simulink model "IEEE34bus_v2019b_Phasor_DPL"  (R2019b)
settings: Solver=VariableStepAuto  StartTime=0.0  StopTime=100  FixedStep=Ts  RelTol=1e-3
InitFcn:
  | a=1; % Loading Factor
  | Ts=0.1;% For Delay Blocks in Voltage Regulator Controls
  | 
  | % Simulation data for the IEEE 34 Node Test Feeder model
  | mi2km = 1.60934;%  miles to km conversion
  | ft2km = 0.0003048; % feet to km conversion
  | ms2F = 1*1e-6/(2*pi*60);% microsiemens to Farads conversion
  | 
  | %% Configuration 300 - series reactance - ohm/mile
  | R_300 = [1.3368 0.2101 0.2130;0.2101 1.3238 0.2066;0.2130 0.2066 1.3294];
  | X_300 = [1.3343 0.5779 0.5015;0.5779 1.3569 0.4591;0.5015 0.4591 1.3471];
  | % charging susceptance - microsiemens/mile
  | B_300 = [5.3350 -1.5313 -0.9943;-1.5313 5.0979 -0.6212;-0.9943 -0.6212 4.8880];
  | 
  | R_300 = R_300/mi2km;
  | L_300 = (X_300/(2*pi*60))/mi2km;
  | C_300 =(B_300*ms2F)/mi2km;
  | 
  | %% Configuration 301 - series reactance - ohm/mile
  | R_301 = [1.9300 0.2327 0.2359;0.2327 1.9157 0.2288;0.2359 0.2288 1.9219];
  | X_301 = [1.4115 0.6442 0.5691;0.6442 1.4281 0.5238;0.5691 0.5238 1.4209];
  | % charging susceptance - microsiemens/mile
  | B_301 = [5.1207 -1.4364 -0.9402;-1.4364 4.9055 -0.5951;-0.9402 -0.5951 4.7154];
  | 
  | R_301 = R_301/mi2km;
  | L_301 = (X_301/(2*pi*60))/mi2km;
  | C_301 =(B_301*ms2F)/mi2km;
  | 
  | 
  | %% Configuration 302 - series reactance - ohm/mile
  | R_302 = [2.7995 0 0;0 0 0;0 0 0];
  | X_302 = [1.4855 0 0;0 0 0;0 0 0];
  | % charging susceptance - microsiemens/mile
  | B_302 = [4.2251 0 0;0 0 0;0 0 0];
  | 
  | R_302 = R_302/mi2km;
  | L_302 = (X_302/(2*pi*60))/mi2km;
  | C_302 =(B_302*ms2F)/mi2km;
  | 
  | %% Configuration 303 - series reactance - ohm/mile
  | R_303 = [0 0 0;0 2.7995 0;0 0 0];
  | X_303 = [0 0 0;0 1.4855 0;0 0 0];
  | % charging susceptance - microsiemens/mile
  | B_303 = [0 0 0;0 4.2251 0;0 0 0];
  | 
  | R_303 = R_303/mi2km;
  | L_303 = (X_303/(2*pi*60))/mi2km;
  | C_303 =(B_303*ms2F)/mi2km;
  | 
  | %% Configuration 303 - series reactance - ohm/mile
  | R_304 = [0 0 0;0 1.9217 0;0 0 0];
  | X_304 = [0 0 0;0 1.4212 0;0 0 0];
  | % charging susceptance - microsiemens/mile
  | B_304 = [0 0 0;0 4.3637 0;0 0 0];
  | 
  | R_304 = R_304/mi2km;
  | L_304 = (X_304/(2*pi*60))/mi2km;
  | C_304 =(B_304*ms2F)/mi2km;
undefined symbols (not defined in the file or in its folder): find_system, j
libraries: powerlib x239, powerlib_meascontrol x22
(part 1 of 4)
settings Model: ARTEMISmethode_block_infos=$$__separator__$$pi34variableloadwith3PV/ARTEMIS Guide$$__separator__$$  Creator=Arun  LastModifiedBy=USARSUR
settings SolverCC: ShapePreserveControl=EnableAll  SolverResetMethod=Robust
settings DataIOCC: ReturnWorkspaceOutputs=off
settings DebuggingCC: UnconnectedInputMsg=none  UnconnectedOutputMsg=none  UnconnectedLineMsg=none  ArithmeticOperatorsInVariantConditions=warning
settings SFSimCC: SimUseLocalCustomCode=off  CustomCodeUndefinedFunction=UseInterfaceOnly
settings RTWCC: RTWUseLocalCustomCode=off
settings CodeAppCC: StateflowObjectComments=on
settings SimscapeCC: SimscapeNormalizeSystem=off

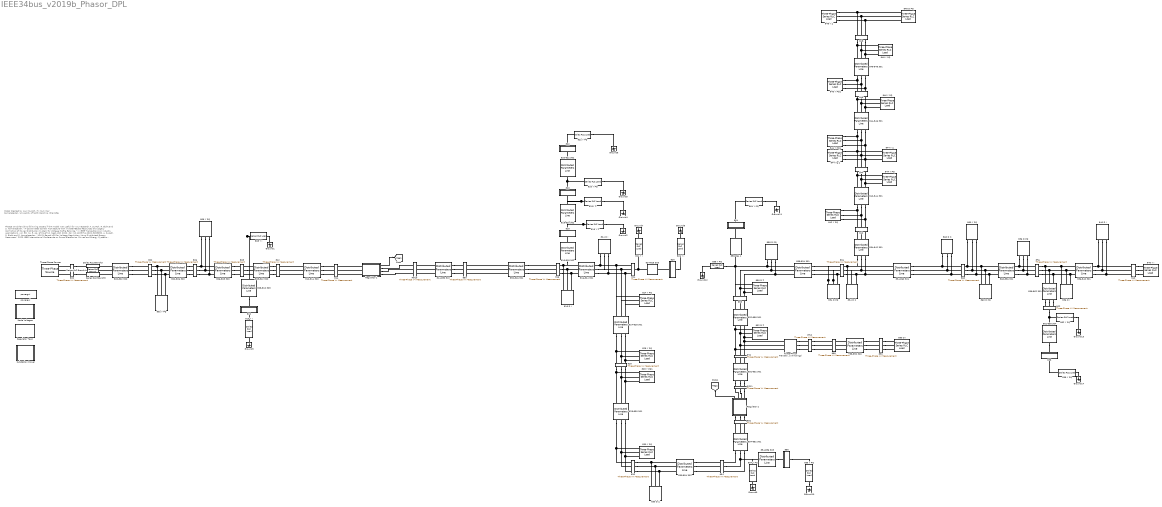
== system IEEE34bus_v2019b_Phasor_DPL ==
  note: Model Created by
      | Arun Suresh, Dr. Sukumar Kamalasadan,
      | University of North Carolina, Charlotte
  note: Please consider citing following papers if the model was useful for your research
      |
      | A. Suresh, R. Bisht and S. Kamalasadan, "A Coordinated Control Architecture With Inverter-Based Resources and Legacy
      | Controllers of Power Distribution System for Voltage Profile Balance," in IEEE Transactions on Industry Applications, vol. 58,
      | no. 5, pp. 6701-6712, Sept.-Oct. 2022, doi: 10.1109/TIA.2022.3183030.
      |
      | A. Suresh, R. Bisht and S. Kamalasadan, "ADMM Based LQR for Voltage Regulation Using Distributed Energy Resources,"
      | 2020 IEEE International Conference on Power Electronics, Drives and Energy Systems (PEDES), 2020, pp. 1-6,
      | doi: 10.1109/PEDES49360.2020.9379625.
  800 : powerlib/Measurements/Three-Phase V-I Measurement  VoltageMeasurement=phase-to-ground  SetLabelV=on  LabelV=V800  Vpu=off  VpuLL=off  CurrentMeasurement=yes  SetLabelI=on  LabelI=I800  Ipu=off  Pbase=100e6  Vbase=24900  OutputType=Complex  PhasorSimulation=on  PSBequivalent=0
      settings: SourceProductName=Simscape Electrical
  800-802 300 : powerlib/Elements/Distributed Parameters Line  Phases=3  Frequency=60  Resistance=R_300  Inductance=L_300  Capacitance=C_300  Length=2580*ft2km  x1=[1249.92473603846 26131.3609955303 26008.9539859825;376.991118430775 376.991118430775 376.991118430775;1.94160409252664 0.298080510916726 1.87234887562591]  x2=[1259.05409163765 26090.5936404474 25972.8081204705;376.991118430775 376.991118430775 376.991118430775;1.94853386735394 0.297367964044877 1.87140996339877]  x3=[10.8891002568441 16.0809137174944 5.85414031081314;376.991118430775 376.991118430775 376.991118430775;1.79537229650244 1.0798554030988 3.0143696476072]  x4=[7.9005802428278 145.280765286366 127.082333761023;376.991118430775 376.991118430775 376.991118430775;-1.40330022719033 0.219032441235353 1.82940682644033]  x5=3.46223763231864e-06  V1=[1250 2.613e+04 2.601e+04;377 377 377;1.942 0.2981 1.872]  V2=[1266 2.604e+04 2.593e+04;377 377 377;1.957 0.2977 1.871]  I1=[20.27 83.58 67.93;377 377 377;1.911 2.489 -2.004]  I2=[17.23 215.7 185.4;377 377 377;-1.237 -0.02332 1.623]  nHarmo=1  Measurements=None
      settings: SourceProductName=Simscape Power Systems
  802 : powerlib/Measurements/Three-Phase V-I Measurement  VoltageMeasurement=phase-to-ground  SetLabelV=on  LabelV=V802  Vpu=off  VpuLL=off  CurrentMeasurement=yes  SetLabelI=on  LabelI=I802  Ipu=off  Pbase=100e6  Vbase=24900  OutputType=Complex  PhasorSimulation=on  PSBequivalent=0
      settings: SourceProductName=Simscape Electrical
  802 Y PQ : powerlib/Elements/Three-Phase Series RLC Load  LConnTagsString=A|B|C  Configuration=Y (grounded)  NominalVoltage=1000  Vabc=[ 1.0 1.0 1.0]*14376.02  Vabcp=[1e3 1e3 1e3]  NominalFrequency=60  UnbalancedPower=on  ActivePower=10e3  InductivePower=100  CapacitivePower=100  Pabc="[1e-3  30 25]*1e3/2 *a"  QLabc=[0 15 14]*1e3/2 *a  QCabc=[0 0 0]  Pabcp=[10e3 9e3 11e3]  QLabcp=[100 90 110]  QCabcp=[100 90 110]  Measurements=None  LoadType=constant PQ
      settings: SourceProductName=Simscape Electrical
  802-806 300 : powerlib/Elements/Distributed Parameters Line  Phases=3  Frequency=60  Resistance=R_300  Inductance=L_300  Capacitance=C_300  Length=1730*ft2km  x1=[1259.05409163765 26090.5936404474 25972.8081204705;376.991118430775 376.991118430775 376.991118430775;1.94896388592436 0.297734464671701 1.87176932780632]  x2=[1265.00206352771 26063.5744788682 25949.4488445243;376.991118430775 376.991118430775 376.991118430775;1.9541920214162 0.297265793458538 1.87113645272041]  x3=[11.3930334018987 16.7161727751993 5.49036931474212;376.991118430775 376.991118430775 376.991118430775;1.8672823424592 1.04909387427718 2.69761493179715]  x4=[8.35366973653815 144.343309301947 125.639738686776;376.991118430775 376.991118430775 376.991118430775;-1.30493901718946 0.217938427430677 1.83893721530045]  x5=2.32157794725242e-06  V1=[1266 2.604e+04 2.593e+04;377 377 377;1.958 0.2981 1.872]  V2=[1276 2.597e+04 2.587e+04;377 377 377;1.969 0.2978 1.871]  I1=[20.86 83.31 66.2;377 377 377;1.948 2.482 -2.001]  I2=[17.78 214.8 183.7;377 377 377;-1.196 -0.02508 1.628]  nHarmo=1  Measurements=None
      settings: SourceProductName=Simscape Power Systems
  806 : powerlib/Measurements/Three-Phase V-I Measurement  VoltageMeasurement=phase-to-ground  SetLabelV=on  LabelV=V806  Vpu=off  VpuLL=off  CurrentMeasurement=yes  SetLabelI=on  LabelI=I806  Ipu=off  Pbase=100e6  Vbase=24900  OutputType=Complex  PhasorSimulation=on  PSBequivalent=0
      settings: SourceProductName=Simscape Electrical
  806 Y PQ : powerlib/Elements/Three-Phase Series RLC Load  LConnTagsString=A|B|C  Configuration=Y (grounded)  NominalVoltage=1000  Vabc=[ 1.0 1.0 1.0]*14376.02  Vabcp=[1e3 1e3 1e3]  NominalFrequency=60  UnbalancedPower=on  ActivePower=10e3  InductivePower=100  CapacitivePower=100  Pabc="[1e-3  30 25]*1e3/2 *a"  QLabc=[0 15 14]*1e3/2 *a  QCabc=[0 0 0]  Pabcp=[10e3 9e3 11e3]  QLabcp=[100 90 110]  QCabcp=[100 90 110]  Measurements=None  LoadType=constant PQ
      settings: SourceProductName=Simscape Electrical
  806-808 300 : powerlib/Elements/Distributed Parameters Line  Phases=3  Frequency=60  Resistance=R_300  Inductance=L_300  Capacitance=C_300  Length=32230*ft2km  x1=[1265.00206352771 26063.5744788682 25949.4488445243;376.991118430775 376.991118430775 376.991118430775;1.93876194330106 0.284114888613696 1.85824161221398]  x2=[1379.02773374669 25564.6834715686 25530.0919618854;376.991118430775 376.991118430775 376.991118430775;2.03883042540818 0.275533008845952 1.84631857982753]  x3=[11.8723696066793 16.932587213612 5.46705259706118;376.991118430775 376.991118430775 376.991118430775;1.91664860231484 1.0200357742312 2.37957123806189]  x4=[8.71372797948738 140.351675369273 121.993071750806;376.991118430775 376.991118430775 376.991118430775;-1.24897193669699 0.190805225356627 1.82267186347869]  x5=4.32511313525697e-05  V1=[1276 2.597e+04 2.587e+04;377 377 377;1.953 0.2847 1.858]  V2=[1495 2.48e+04 2.487e+04;377 377 377;2.136 0.2802 1.845]  I1=[21.34 82.37 64.1;377 377 377;1.967 2.465 -2.009]  I2=[18.04 208.6 178.4;377 377 377;-1.188 -0.05185 1.608]  nHarmo=1  Measurements=None
      settings: SourceProductName=Simscape Power Systems
  808 : powerlib/Measurements/Three-Phase V-I Measurement  VoltageMeasurement=phase-to-ground  SetLabelV=on  LabelV=V808  Vpu=off  VpuLL=off  CurrentMeasurement=yes  SetLabelI=on  LabelI=I808  Ipu=off  Pbase=100e6  Vbase=24900  OutputType=Complex  PhasorSimulation=on  PSBequivalent=0
      settings: SourceProductName=Simscape Electrical
  808 Y I : powerlib/Elements/Series RLC Load  LConnTagsString=a  RConnTagsString=__new0  NominalVoltage=1.0*14376.02  NominalFrequency=60  ActivePower=16e3/2*a  InductivePower=8e3/2*a  CapacitivePower=0  Setx0=off  InitialVoltage=0  SetiL0=off  InitialCurrent=0  Measurements=None  LoadType=constant I
      settings: SourceProductName=Simscape Electrical
  808-810 303 : powerlib/Elements/Distributed Parameters Line  Phases=1  Frequency=60  Resistance=R_303(2,2)  Inductance=L_303(2,2)  Capacitance=C_303(2,2)  Length=5804*ft2km  x1=[20983.741763622;376.991118430775;-2.11327141774278]  x2=[20980.659007782;376.991118430775;-2.11328221150665]  x3=[34.4426323640272;376.991118430775;-2.10433384251084]  x4=[36.0584227611352;376.991118430775;-2.12451473195879]  x5=7.30496713110932e-06  V1=[2.049e+04;377;-2.115]  V2=[2.048e+04;377;-2.115]  I1=[33.62;377;-2.106]  I2=[35.2;377;-2.126]  nHarmo=1  Measurements=None
      settings: SourceProductName=Simscape Power Systems
  808-812 300 : powerlib/Elements/Distributed Parameters Line  Phases=3  Frequency=60  Resistance=R_300  Inductance=L_300  Capacitance=C_300  Length=37500*ft2km  x1=[1379.02773374669 25564.6834715686 25530.0919618854;376.991118430775 376.991118430775 376.991118430775;2.03616431027156 0.273260704959647 1.84409052050068]  x2=[1508.53935989797 24986.4688915968 25049.8377706755;376.991118430775 376.991118430775 376.991118430775;2.14075084651696 0.263537048880938 1.82978913917078]  x3=[11.7784392805967 17.0338463877836 4.39298540674719;376.991118430775 376.991118430775 376.991118430775;2.01811649155585 1.07121274431336 2.29220318868309]  x4=[8.3337594581597 137.573158671839 120.282432485824;376.991118430775 376.991118430775 376.991118430775;-1.14964617525409 0.170446005290606 1.81272355740158]  x5=5.03232213999802e-05  V1=[1495 2.48e+04 2.487e+04;377 377 377;2.133 0.2779 1.843]  V2=[1780 2.344e+04 2.372e+04;377 377 377;2.292 0.2729 1.827]  I1=[21.39 84.55 65.08;377 377 377;2.029 2.481 -1.979]  I2=[17.55 204.1 175.2;377 377 377;-1.153 -0.07064 1.596]  nHarmo=1  Measurements=None
      settings: SourceProductName=Simscape Power Systems
  810 : Subsystem
  810 Y I : powerlib/Elements/Series RLC Load  LConnTagsString=a  RConnTagsString=__new0  NominalVoltage=1.0*14376.02  NominalFrequency=60  ActivePower=16e3/2*a  InductivePower=8e3/2*a  CapacitivePower=0  Setx0=off  InitialVoltage=0  SetiL0=off  InitialCurrent=0  Measurements=None  LoadType=constant I
      settings: SourceProductName=Simscape Electrical
  812 : powerlib/Measurements/Three-Phase V-I Measurement  VoltageMeasurement=phase-to-ground  SetLabelV=on  LabelV=V812  Vpu=off  VpuLL=off  CurrentMeasurement=yes  SetLabelI=on  LabelI=I812  Ipu=off  Pbase=100e6  Vbase=24900  OutputType=Complex  PhasorSimulation=on  PSBequivalent=0
      settings: SourceProductName=Simscape Electrical
  812-814 300 : powerlib/Elements/Distributed Parameters Line  Phases=3  Frequency=60  Resistance=R_300  Inductance=L_300  Capacitance=C_300  Length=29730*ft2km  x1=[1508.53935989797 24986.4688915968 25049.8377706755;376.991118430775 376.991118430775 376.991118430775;2.14468172215481 0.266887295787312 1.8330741526375]  x2=[1620.85281381877 24525.100342828 24668.3082857637;376.991118430775 376.991118430775 376.991118430775;2.21533373989356 0.25913080618959 1.82156491116368]  x3=[11.9386409643217 16.3733340285274 3.49017953051114;376.991118430775 376.991118430775 376.991118430775;2.04085486735346 1.16632302809471 2.46326904583715]  x4=[8.23217709885128 136.789856752813 119.676212236204;376.991118430775 376.991118430775 376.991118430775;-1.1612015700944 0.161983892125807 1.80358561310401]  x5=3.98962499259043e-05  V1=[1780 2.344e+04 2.372e+04;377 377 377;2.296 0.2763 1.83]  V2=[2029 2.235e+04 2.281e+04;377 377 377;2.389 0.2721 1.816]  I1=[21.69 87.78 67.39;377 377 377;2.051 2.515 -1.95]  I2=[17.36 202.1 173.8;377 377 377;-1.165 -0.07782 1.588]  nHarmo=1  Measurements=None
      settings: SourceProductName=Simscape Power Systems
  814 : powerlib/Measurements/Three-Phase V-I Measurement  VoltageMeasurement=phase-to-ground  SetLabelV=on  LabelV=V814  Vpu=off  VpuLL=off  CurrentMeasurement=yes  SetLabelI=on  LabelI=I814  Ipu=off  Pbase=100e6  Vbase=24900  OutputType=Complex  PhasorSimulation=on  PSBequivalent=0
      settings: SourceProductName=Simscape Electrical
  814-850 301 : powerlib/Elements/Distributed Parameters Line  Phases=3  Frequency=60  Resistance=R_301  Inductance=L_301  Capacitance=C_301  Length=10*ft2km  x1=[541.716185552378 24529.7060586551 24692.5777448304;376.991118430775 376.991118430775 376.991118430775;-1.38184455477449 0.270413103653491 1.8310302394934]  x2=[541.683717853495 24529.4812379324 24692.3879781101;376.991118430775 376.991118430775 376.991118430775;-1.38196447318103 0.270411019646005 1.83102646637729]  x3=[10.6293599098107 15.0605983819621 2.72613552566952;376.991118430775 376.991118430775 376.991118430775;2.05835663684987 1.34412851974194 2.80869119845773]  x4=[11.7651518062053 136.309982115356 118.387556519995;376.991118430775 376.991118430775 376.991118430775;-1.11282793802951 0.173140030599462 1.8119310704332]  x5=1.37899021776565e-08  V1=[322.2 2.375e+04 2.363e+04;377 377 377;-1.555 0.2746 1.834]  V2=[322.1 2.375e+04 2.363e+04;377 377 377;-1.555 0.2746 1.834]  I1=[17.89 80.08 64.4;377 377 377;1.9 2.507 -1.985]  I2=[18.56 197.9 169.8;377 377 377;-1.253 -0.05041 1.594]  nHarmo=1  Measurements=None
      settings: SourceProductName=Simscape Power Systems
  "816 " : powerlib/Measurements/Three-Phase V-I Measurement  VoltageMeasurement=phase-to-ground  SetLabelV=on  LabelV=V816  Vpu=off  VpuLL=off  CurrentMeasurement=yes  SetLabelI=on  LabelI=I816  Ipu=off  Pbase=100e6  Vbase=24900  OutputType=Complex  PhasorSimulation=on  PSBequivalent=0
      settings: SourceProductName=Simscape Electrical
  816 D I : powerlib/Elements/Three-Phase Series RLC Load  LConnTagsString=A|B|C  Configuration=Delta  NominalVoltage=1000  Vabc=[1e3 1e3 1e3]  Vabcp=[ 1.0 1.0 1.0]*24900  NominalFrequency=60  UnbalancedPower=on  ActivePower=10e3  InductivePower=100  CapacitivePower=100  Pabc=[10e3 9e3 11e3]  QLabc=[100 90 110]  QCabc=[100 90 110]  Pabcp="[1e-3  5 1e-3 ]*1e3/2 *a"  QLabcp=[0 2 0]*1e3/2 *a  QCabcp=[0 0 0]  Measurements=None  LoadType=constant I
      settings: SourceProductName=Simscape Electrical
  816-818 302 : powerlib/Elements/Distributed Parameters Line  Phases=1  Frequency=60  Resistance=R_302(1,1)  Inductance=L_302(1,1)  Capacitance=C_302(1,1)  Length=1710*ft2km  x1=[19599.043291833;376.991118430775;-0.0276711309327301]  x2=[19581.4286914405;376.991118430775;-0.0277266237467162]  x3=[18.762900155392;376.991118430775;0.359835239332487]  x4=[49.1480740831425;376.991118430775;-0.173025484635906]  x5=2.15222153587128e-06  V1=[1.888e+04;377;-0.01414]  V2=[1.887e+04;377;-0.01419]  I1=[18.08;377;0.3734]  I2=[47.35;377;-0.1595]  nHarmo=1  Measurements=None
      settings: SourceProductName=Simscape Power Systems
  816-824 301 : powerlib/Elements/Distributed Parameters Line  Phases=3  Frequency=60  Resistance=R_301  Inductance=L_301  Capacitance=C_301  Length=10210*ft2km  x1=[540.68108300544 24522.5116299881 24686.5051711599;376.991118430775 376.991118430775 376.991118430775;-1.39099170085732 0.266024838739706 1.82665567930449]  x2=[494.892872188634 24338.1699053478 24496.4148193842;376.991118430775 376.991118430775 376.991118430775;-1.38678289131807 0.263343360345804 1.8233381768605]  x3=[6.5395647034292 17.4484669356444 6.37351923620024;376.991118430775 376.991118430775 376.991118430775;0.812338222813492 0.529487155526738 2.71916510612684]  x4=[7.26322004074914 124.514374907441 114.823791238699;376.991118430775 376.991118430775 376.991118430775;-2.20387956309574 0.225544955070776 1.77950460460417]  x5=1.40794901233873e-05  V1=[320.6 2.373e+04 2.361e+04;377 377 377;-1.571 0.2704 1.83]  V2=[250.1 2.33e+04 2.32e+04;377 377 377;-1.761 0.2712 1.828]  I1=[13.01 67.52 63.68;377 377 377;1.303 2.466 -2.045]  I2=[13.62 183.9 166;377 377 377;-1.831 -0.03341 1.568]  nHarmo=1  Measurements=None
      settings: SourceProductName=Simscape Power Systems
  818 : Subsystem
  818 Y Z : powerlib/Elements/Series RLC Load  LConnTagsString=a  RConnTagsString=__new0  NominalVoltage=1.0*14376.02  NominalFrequency=60  ActivePower=34e3/2 *a  InductivePower=17e3/2*a  CapacitivePower=0  Setx0=off  InitialVoltage=0  SetiL0=off  InitialCurrent=0  Measurements=None  LoadType=constant Z
      settings: SourceProductName=Simscape Electrical
  818-820 302 : powerlib/Elements/Distributed Parameters Line  Phases=1  Frequency=60  Resistance=R_302(1,1)  Inductance=L_302(1,1)  Capacitance=C_302(1,1)  Length=48150*ft2km  x1=[19581.4286914405;376.991118430775;-0.0497616814531457]  x2=[19132.2355748454;376.991118430775;-0.050779558971269]  x3=[19.2494034235055;376.991118430775;0.277164280556863]  x4=[45.5212647504315;376.991118430775;-0.202890199688713]  x5=6.06020274574283e-05  V1=[1.887e+04;377;-0.03623]  V2=[1.843e+04;377;-0.03725]  I1=[18.55;377;0.2907]  I2=[43.86;377;-0.1894]  nHarmo=1  Measurements=None
      settings: SourceProductName=Simscape Power Systems
  820 : Subsystem
  820 Y PQ : powerlib/Elements/Series RLC Load  LConnTagsString=a  RConnTagsString=__new0  NominalVoltage=1.0*14376.02  NominalFrequency=60  ActivePower=135e3/2 *a  InductivePower=70e3/2*a  CapacitivePower=0  Setx0=off  InitialVoltage=0  SetiL0=off  InitialCurrent=0  Measurements=None  LoadType=constant PQ
      settings: SourceProductName=Simscape Electrical
  820-822 302 : powerlib/Elements/Distributed Parameters Line  Phases=1  Frequency=60  Resistance=R_302(1,1)  Inductance=L_302(1,1)  Capacitance=C_302(1,1)  Length=13740*ft2km  x1=[19132.2355748454;376.991118430775;-0.034452549159076]  x2=[19074.7680195885;376.991118430775;-0.0345212563962167]  x3=[25.9530323871068;376.991118430775;0.0814867359847224]  x4=[38.2013347778514;376.991118430775;-0.118663890946888]  x5=1.72932888320886e-05  V1=[1.843e+04;377;-0.02092]  V2=[1.838e+04;377;-0.02099]  I1=[25.01;377;0.09502]  I2=[36.81;377;-0.1051]  nHarmo=1  Measurements=None
      settings: SourceProductName=Simscape Power Systems
  820Y Z : powerlib/Elements/Series RLC Load  LConnTagsString=a  RConnTagsString=__new0  NominalVoltage=1.0*14376.02  NominalFrequency=60  ActivePower=34e3/2 *a  InductivePower=17e3/2*a  CapacitivePower=0  Setx0=off  InitialVoltage=0  SetiL0=off  InitialCurrent=0  Measurements=None  LoadType=constant Z
      settings: SourceProductName=Simscape Electrical
  822 : Subsystem
  822 Y PQ : powerlib/Elements/Series RLC Load  LConnTagsString=a  RConnTagsString=__new0  NominalVoltage=1.0*14376.02  NominalFrequency=60  ActivePower=135e3/2*a  InductivePower=70e3/2*a  CapacitivePower=0  Setx0=off  InitialVoltage=0  SetiL0=off  InitialCurrent=0  Measurements=None  LoadType=constant PQ
      settings: SourceProductName=Simscape Electrical
  "824 " : powerlib/Measurements/Three-Phase V-I Measurement  VoltageMeasurement=phase-to-ground  SetLabelV=on  LabelV=V824  Vpu=off  VpuLL=off  CurrentMeasurement=yes  SetLabelI=on  LabelI=I824  Ipu=off  Pbase=100e6  Vbase=24900  OutputType=Complex  PhasorSimulation=on  PSBequivalent=0
      settings: SourceProductName=Simscape Electrical
  824 D I : powerlib/Elements/Three-Phase Series RLC Load  LConnTagsString=A|B|C  Configuration=Delta  NominalVoltage=1000  Vabc=[1e3 1e3 1e3]  Vabcp=[ 1.0 1.0 1.0]*24900  NominalFrequency=60  UnbalancedPower=on  ActivePower=10e3  InductivePower=100  CapacitivePower=100  Pabc=[10e3 9e3 11e3]  QLabc=[100 90 110]  QCabc=[100 90 110]  Pabcp="[1e-3  5 1e-3] *1e3/2 *a"  QLabcp=[0 2 0]*1e3/2 *a  QCabcp=[0 0 0]  Measurements=None  LoadType=constant I
      settings: SourceProductName=Simscape Electrical
  824 Y I : powerlib/Elements/Series RLC Load  LConnTagsString=a  RConnTagsString=__new0  NominalVoltage=1.0*14376.02  NominalFrequency=60  ActivePower=40e3/2 *a  InductivePower=20e3/2*a  CapacitivePower=0  Setx0=off  InitialVoltage=0  SetiL0=off  InitialCurrent=0  Measurements=None  LoadType=constant I
      settings: SourceProductName=Simscape Electrical
  824 Y PQ : powerlib/Elements/Three-Phase Series RLC Load  LConnTagsString=A|B|C  Configuration=Y (grounded)  NominalVoltage=1000  Vabc=[ 1.0 1.0 1.0]*14376.02  Vabcp=[1e3 1e3 1e3]  NominalFrequency=60  UnbalancedPower=on  ActivePower=10e3  InductivePower=100  CapacitivePower=100  Pabc="[1e-3  1e-3  4]*1e3/2 *a"  QLabc=[0 0 2]*1e3/2 *a  QCabc=[0 0 0]  Pabcp=[10e3 9e3 11e3]  QLabcp=[100 90 110]  QCabcp=[100 90 110]  Measurements=None  LoadType=constant PQ
      settings: SourceProductName=Simscape Electrical
  824-826 303 : powerlib/Elements/Distributed Parameters Line  Phases=1  Frequency=60  Resistance=R_303(2,2)  Inductance=L_303(2,2)  Capacitance=C_303(2,2)  Length=3030*ft2km  x1=[20193.9369942493;376.991118430775;-2.1452384534769]  x2=[20189.9861498664;376.991118430775;-2.14524516202024]  x3=[32.0498339340208;376.991118430775;-2.11631951694802]  x4=[35.9454061074803;376.991118430775;-2.1723895644908]  x5=3.81358552847368e-06  V1=[1.921e+04;377;-2.151]  V2=[1.92e+04;377;-2.151]  I1=[30.48;377;-2.122]  I2=[34.19;377;-2.179]  nHarmo=1  Measurements=None
      settings: SourceProductName=Simscape Power Systems
  824-828 301 : powerlib/Elements/Distributed Parameters Line  Phases=3  Frequency=60  Resistance=R_301  Inductance=L_301  Capacitance=C_301  Length=840*ft2km  x1=[494.892872188636 24338.1699053478 24496.4148193842;376.991118430775 376.991118430775 376.991118430775;-1.3819117369237 0.26731327988838 1.82724584136767]  x2=[492.386131641842 24323.596825107 24481.3827649556;376.991118430775 376.991118430775 376.991118430775;-1.38270611551351 0.26711380783541 1.82695166941058]  x3=[4.24529447419059 19.8772094474859 5.3392961228501;376.991118430775 376.991118430775 376.991118430775;1.01126091496231 0.545527859778125 2.34420034312088]  x4=[5.08852546976801 122.618552452885 114.233921208007;376.991118430775 376.991118430775 376.991118430775;-1.98580061545121 0.222456849721216 1.80380791469247]  x5=1.15835178292315e-06  V1=[250.1 2.33e+04 2.32e+04;377 377 377;-1.756 0.2751 1.832]  V2=[246.2 2.326e+04 2.317e+04;377 377 377;-1.777 0.2752 1.831]  I1=[11.57 67.9 62.08;377 377 377;1.466 2.443 -2.015]  I2=[12.11 182.5 164.8;377 377 377;-1.679 -0.03759 1.585]  nHarmo=1  Measurements=None
      settings: SourceProductName=Simscape Power Systems
  826 : Subsystem
  826 Y I : powerlib/Elements/Series RLC Load  LConnTagsString=a  RConnTagsString=__new0  NominalVoltage=1.0*14376.02  NominalFrequency=60  ActivePower=40e3/2 *a  InductivePower=20e3/2*a  CapacitivePower=0  Setx0=off  InitialVoltage=0  SetiL0=off  InitialCurrent=0  Measurements=None  LoadType=constant I
      settings: SourceProductName=Simscape Electrical
  828 : powerlib/Measurements/Three-Phase V-I Measurement  VoltageMeasurement=phase-to-ground  SetLabelV=on  LabelV=V828  Vpu=off  VpuLL=off  CurrentMeasurement=yes  SetLabelI=on  LabelI=I828  Ipu=off  Pbase=100e6  Vbase=24900  OutputType=Complex  PhasorSimulation=on  PSBequivalent=0
      settings: SourceProductName=Simscape Electrical
  828 Y PQ : powerlib/Elements/Three-Phase Series RLC Load  LConnTagsString=A|B|C  Configuration=Y (grounded)  NominalVoltage=1000  Vabc=[ 1.0 1.0 1.0]*14376.02  Vabcp=[1e3 1e3 1e3]  NominalFrequency=60  UnbalancedPower=on  ActivePower=10e3  InductivePower=100  CapacitivePower=100  Pabc="[1e-3  1e-3  4]*1e3/2 *a"  QLabc=[0 0 2]*1e3/2 *a  QCabc=[0 0 0]  Pabcp=[10e3 9e3 11e3]  QLabcp=[100 90 110]  QCabcp=[100 90 110]  Measurements=None  LoadType=constant PQ
      settings: SourceProductName=Simscape Electrical
  828 Y PQ1 : powerlib/Elements/Three-Phase Series RLC Load  LConnTagsString=A|B|C  Configuration=Y (grounded)  NominalVoltage=1000  Vabc=[ 1.0 1.0 1.0]*14376.02  Vabcp=[1e3 1e3 1e3]  NominalFrequency=60  UnbalancedPower=on  ActivePower=10e3  InductivePower=100  CapacitivePower=100  Pabc="[7 1e-3  1e-3 ]*1e3/2 *a"  QLabc=[3 0 0]*1e3/2 *a  QCabc=[0 0 0]  Pabcp=[10e3 9e3 11e3]  QLabcp=[100 90 110]  QCabcp=[100 90 110]  Measurements=None  LoadType=constant PQ
      settings: SourceProductName=Simscape Electrical
  828-830 301 : powerlib/Elements/Distributed Parameters Line  Phases=3  Frequency=60  Resistance=R_301  Inductance=L_301  Capacitance=C_301  Length=20440*ft2km  x1=[492.386131641842 24323.596825107 24481.3827649556;376.991118430775 376.991118430775 376.991118430775;-1.39289550997772 0.258809600467803 1.81877768602311]  x2=[429.60597370121 23970.2991285525 24116.7232197737;376.991118430775 376.991118430775 376.991118430775;-1.41073727108047 0.253933225552265 1.81161565049166]  x3=[4.35662309388594 19.4844448394639 5.27978481404586;376.991118430775 376.991118430775 376.991118430775;0.967084996782615 0.529382604566783 2.34312152823618]  x4=[5.12273487844301 120.007143283172 112.075052811202;376.991118430775 376.991118430775 376.991118430775;-2.03857052511841 0.207569220220189 1.78703850540164]  x5=2.81865600511299e-05  V1=[246.2 2.326e+04 2.317e+04;377 377 377;-1.787 0.2669 1.823]  V2=[194.3 2.24e+04 2.235e+04;377 377 377;-2.482 0.2693 1.819]  I1=[11.57 67.26 61.69;377 377 377;1.441 2.439 -2.023]  I2=[11.98 178.1 161.4;377 377 377;-1.715 -0.05215 1.569]  nHarmo=1  Measurements=None
      settings: SourceProductName=Simscape Power Systems
  830 : powerlib/Measurements/Three-Phase V-I Measurement  VoltageMeasurement=phase-to-ground  SetLabelV=on  LabelV=V830  Vpu=off  VpuLL=off  CurrentMeasurement=no  SetLabelI=on  LabelI=I830  Ipu=off  Pbase=100e6  Vbase=24900  OutputType=Complex  PhasorSimulation=on  PSBequivalent=0
      settings: SourceProductName=Simscape Electrical
  830 D Z : powerlib/Elements/Three-Phase Series RLC Load  LConnTagsString=A|B|C  Configuration=Delta  NominalVoltage=1000  Vabc=[1e3 1e3 1e3]  Vabcp=[ 1.0 1.0 1.0]*24900  NominalFrequency=60  UnbalancedPower=on  ActivePower=10e3  InductivePower=100  CapacitivePower=100  Pabc=[10e3 9e3 11e3]  QLabc=[100 90 110]  QCabc=[100 90 110]  Pabcp=[10 10 25]*1e3 *a  QLabcp=[5 5 10]*1e3 *a  QCabcp=[0 0 0]  Measurements=None  LoadType=constant Z
      settings: SourceProductName=Simscape Electrical
  830 Y PQ : powerlib/Elements/Three-Phase Series RLC Load  LConnTagsString=A|B|C  Configuration=Y (grounded)  NominalVoltage=1000  Vabc=[ 1.0 1.0 1.0]*14376.02  Vabcp=[1e3 1e3 1e3]  NominalFrequency=60  UnbalancedPower=on  ActivePower=10e3  InductivePower=100  CapacitivePower=100  Pabc="[7 1e-3  1e-3 ]*1e3/2 *a"  QLabc=[3 0 0]*1e3/2 *a  QCabc=[0 0 0]  Pabcp=[10e3 9e3 11e3]  QLabcp=[100 90 110]  QCabcp=[100 90 110]  Measurements=None  LoadType=constant PQ
      settings: SourceProductName=Simscape Electrical
  830-854 301 : powerlib/Elements/Distributed Parameters Line  Phases=3  Frequency=60  Resistance=R_301  Inductance=L_301  Capacitance=C_301  Length=520*ft2km  x1=[429.60597370121 23970.2991285525 24116.7232197737;376.991118430775 376.991118430775 376.991118430775;-1.40038151915561 0.26237301181567 1.81992308666913]  x2=[428.013916342019 23961.6924006652 24107.7905484182;376.991118430775 376.991118430775 376.991118430775;-1.40064933945479 0.262244139729698 1.81974626756815]  x3=[4.40100643252979 20.3428500290921 6.51245170311381;376.991118430775 376.991118430775 376.991118430775;0.916037803689389 0.46556461510103 2.23316970510581]  x4=[5.08314125552688 119.662529256945 111.105093726173;376.991118430775 376.991118430775 376.991118430775;-2.08984862029727 0.227856854384458 1.79617452197055]  x5=7.17074913238139e-07  V1=[194.3 2.24e+04 2.235e+04;377 377 377;-2.471 0.2778 1.827]  V2=[194.3 2.238e+04 2.233e+04;377 377 377;-2.491 0.2778 1.827]  I1=[11.39 64.06 59.1;377 377 377;1.429 2.447 -2.052]  I2=[11.7 174.7 157.3;377 377 377;-1.738 -0.03018 1.572]  nHarmo=1  Measurements=None
      settings: SourceProductName=Simscape Power Systems
  832 : powerlib/Measurements/Three-Phase V-I Measurement  VoltageMeasurement=phase-to-ground  SetLabelV=on  LabelV=V832  Vpu=off  VpuLL=off  CurrentMeasurement=no  SetLabelI=off  LabelI=I815  Ipu=off  Pbase=100e6  Vbase=24900  OutputType=Complex  PhasorSimulation=on  PSBequivalent=0
      settings: SourceProductName=Simscape Electrical
  832 D Z : powerlib/Elements/Three-Phase Series RLC Load  LConnTagsString=A|B|C  Configuration=Delta  NominalVoltage=1000  Vabc=[1e3 1e3 1e3]  Vabcp=[ 1.0 1.0 1.0]*24900  NominalFrequency=60  UnbalancedPower=on  ActivePower=10e3  InductivePower=100  CapacitivePower=100  Pabc=[10e3 9e3 11e3]  QLabc=[100 90 110]  QCabc=[100 90 110]  Pabcp=[7 2 6]*1e3/2 *a  QLabcp=[3 1 3]*1e3/2*a  QCabcp=[0 0 0]  Measurements=None  LoadType=constant Z
      settings: SourceProductName=Simscape Electrical
  832-858 301 : powerlib/Elements/Distributed Parameters Line  Phases=3  Frequency=60  Resistance=R_301  Inductance=L_301  Capacitance=C_301  Length=4900*ft2km  x1=[320.48155576948 23349.9161493877 23477.0352904044;376.991118430775 376.991118430775 376.991118430775;-1.41897084797957 0.251435923296132 1.80528986204469]  x2=[308.059778746511 23297.1351077948 23423.0500557617;376.991118430775 376.991118430775 376.991118430775;-1.41532043160503 0.250130065954545 1.80356009180675]  x3=[3.71706926690036 32.8013458512137 20.0348811764682;376.991118430775 376.991118430775 376.991118430775;0.733727973159427 0.146027381116314 1.51760725983672]  x4=[4.13317790449903 102.791779194849 94.4820808895792;376.991118430775 376.991118430775 376.991118430775;-2.26889031503577 0.282787862808818 1.86322019256521]  x5=6.7570520670517e-06  V1=[606 2.261e+04 2.152e+04;377 377 377;-1.527 0.2929 1.805]  V2=[590 2.25e+04 2.141e+04;377 377 377;-1.536 0.2932 1.803]  I1=[4.722 32.22 18.38;377 377 377;1.035 1.566 -2.28]  I2=[5.86 125.4 115.7;377 377 377;-1.986 0.04361 1.674]  nHarmo=1  Measurements=None
      settings: SourceProductName=Simscape Power Systems
  834 : powerlib/Measurements/Three-Phase V-I Measurement  VoltageMeasurement=phase-to-ground  SetLabelV=on  LabelV=V834  Vpu=off  VpuLL=off  CurrentMeasurement=yes  SetLabelI=on  LabelI=I834  Ipu=off  Pbase=100e6  Vbase=24900  OutputType=Complex  PhasorSimulation=on  PSBequivalent=0
      settings: SourceProductName=Simscape Electrical
  834 D PQ : powerlib/Elements/Three-Phase Series RLC Load  LConnTagsString=A|B|C  Configuration=Delta  NominalVoltage=[ 1.0 1.0 1.0]*2401.78  Vabc=[1e3 1e3 1e3]  Vabcp=[ 1.0 1.0 1.0]*24900  NominalFrequency=60  UnbalancedPower=on  ActivePower=[4 15 13]*1e3/2  InductivePower=[2 8 7]*1e3/2  CapacitivePower=100  Pabc=[10e3 9e3 11e3]  QLabc=[100 90 110]  QCabc=[100 90 110]  Pabcp=[4 15 13]*1e3/2 *a  QLabcp=[2 8 7]*1e3/2 *a  QCabcp=[0 0 0]  Measurements=None  LoadType=constant PQ
      settings: SourceProductName=Simscape Electrical
  834 D Z : powerlib/Elements/Three-Phase Series RLC Load  LConnTagsString=A|B|C  Configuration=Delta  NominalVoltage=1000  Vabc=[1e3 1e3 1e3]  Vabcp=[ 1.0 1.0 1.0]*24900  NominalFrequency=60  UnbalancedPower=on  ActivePower=10e3  InductivePower=100  CapacitivePower=100  Pabc=[10e3 9e3 11e3]  QLabc=[100 90 110]  QCabc=[100 90 110]  Pabcp=[16 20 110]*1e3/2 *a  QLabcp=[8 10 55]*1e3/2 *a  QCabcp=[0 0 0]  Measurements=None  LoadType=constant Z
      settings: SourceProductName=Simscape Electrical
  834-842 301 : powerlib/Elements/Distributed Parameters Line  Phases=3  Frequency=60  Resistance=R_301  Inductance=L_301  Capacitance=C_301  Length=280*ft2km  x1=[293.318135105792 23236.3015016255 23361.1779978373;376.991118430775 376.991118430775 376.991118430775;-1.40615135501835 0.250524945746872 1.80344226509278]  x2=[292.992794774887 23235.0415061901 23359.9419144581;376.991118430775 376.991118430775 376.991118430775;-1.40577311642595 0.250432255295562 1.80335512629569]  x3=[1.78640744473078 49.1597223244208 38.3037520411461;376.991118430775 376.991118430775 376.991118430775;0.418431352103275 -0.0514709338681054 1.4877381001421]  x4=[2.04329075546246 89.5511403743045 77.9057441453781;376.991118430775 376.991118430775 376.991118430775;-2.41503748204938 0.414371701140957 1.95654725775113]  x5=3.86117260974383e-07  V1=[571.2 2.238e+04 2.128e+04;377 377 377;-1.543 0.2956 1.803]  V2=[570.8 2.237e+04 2.128e+04;377 377 377;-1.543 0.2956 1.803]  I1=[2.103 40.93 29.58;377 377 377;0.4778 0.3685 1.992]  I2=[2.874 89.51 74.48;377 377 377;-2.263 0.2622 1.729]  nHarmo=1  Measurements=None
      settings: SourceProductName=Simscape Power Systems
  834-860 301 : powerlib/Elements/Distributed Parameters Line  Phases=3  Frequency=60  Resistance=R_301  Inductance=L_301  Capacitance=C_301  Length=2020*ft2km  x1=[293.318135105792 23236.3015016255 23361.1779978373;376.991118430775 376.991118430775 376.991118430775;-1.40705592371059 0.249787735500972 1.80271661554716]  x2=[290.754060428224 23226.5580690742 23351.6426236293;376.991118430775 376.991118430775 376.991118430775;-1.40620080248349 0.249852317045646 1.80270250705443]  x3=[1.78964859406605 56.4663524839272 45.3239762071133;376.991118430775 376.991118430775 376.991118430775;0.670900155348255 0.384210807134 1.9305216996231]  x4=[2.17189959496333 79.5068776325778 68.564360773579;376.991118430775 376.991118430775 376.991118430775;-2.21130738958258 0.153786762395425 1.71765146592785]  x5=2.78556023988662e-06  V1=[571.2 2.238e+04 2.128e+04;377 377 377;-1.544 0.2949 1.803]  V2=[568.3 2.236e+04 2.127e+04;377 377 377;-1.546 0.2951 1.803]  I1=[1.883 44.84 27.82;377 377 377;1.013 0.7038 2.104]  I2=[3.001 90.71 77.07;377 377 377;-1.898 0.0966 1.695]  nHarmo=1  Measurements=None
      settings: SourceProductName=Simscape Power Systems
  836 : powerlib/Measurements/Three-Phase V-I Measurement  VoltageMeasurement=phase-to-ground  SetLabelV=on  LabelV=V836  Vpu=off  VpuLL=off  CurrentMeasurement=yes  SetLabelI=on  LabelI=I836  Ipu=off  Pbase=100e6  Vbase=24900  OutputType=Complex  PhasorSimulation=on  PSBequivalent=0
      settings: SourceProductName=Simscape Electrical
  836 D I : powerlib/Elements/Three-Phase Series RLC Load  LConnTagsString=A|B|C  Configuration=Delta  NominalVoltage=1000  Vabc=[1e3 1e3 1e3]  Vabcp=[ 1.0 1.0 1.0]*24900  NominalFrequency=60  UnbalancedPower=on  ActivePower=10e3  InductivePower=100  CapacitivePower=100  Pabc=[10e3 9e3 11e3]  QLabc=[100 90 110]  QCabc=[100 90 110]  Pabcp=[18 22 1e-3 ]*1e3/2 *a  QLabcp=[9 11 0]*1e3/2 *a  QCabcp=[0 0 0]  Measurements=None  LoadType=constant I
      settings: SourceProductName=Simscape Electrical
  836 D PQ : powerlib/Elements/Three-Phase Series RLC Load  LConnTagsString=A|B|C  Configuration=Delta  NominalVoltage=1000  Vabc=[1e3 1e3 1e3]  Vabcp=[ 1.0 1.0 1.0]*24900  NominalFrequency=60  UnbalancedPower=on  ActivePower=10e3  InductivePower=100  CapacitivePower=100  Pabc=[10e3 9e3 11e3]  QLabc=[100 90 110]  QCabc=[100 90 110]  Pabcp=[30 10 42]*1e3/2 *a  QLabcp=[15 6 22]*1e3/2 *a  QCabcp=[0 0 0]  Measurements=None  LoadType=constant Z
      settings: SourceProductName=Simscape Electrical
  836-840 301 : powerlib/Elements/Distributed Parameters Line  Phases=3  Frequency=60  Resistance=R_301  Inductance=L_301  Capacitance=C_301  Length=860*ft2km  x1=[287.744791807787 23220.7079462666 23346.2225579365;376.991118430775 376.991118430775 376.991118430775;-1.40248380825547 0.250297804337013 1.80325122468632]  x2=[287.711040346335 23220.0845595466 23345.5429949187;376.991118430775 376.991118430775 376.991118430775;-1.40251725270496 0.250296298318595 1.80325930388645]  x3=[0.262397773687727 65.652239749222 55.036622378366;376.991118430775 376.991118430775 376.991118430775;-1.27785402091571 0.261504747361211 1.83162259195034]  x4=[0.369268749369741 69.4991069477184 58.302776117434;376.991118430775 376.991118430775 376.991118430775;-1.49134074182044 0.239355385990802 1.77612882231741]  x5=1.18593158727846e-06  V1=[565 2.234e+04 2.126e+04;377 377 377;-1.546 0.2955 1.803]  V2=[564.9 2.234e+04 2.125e+04;377 377 377;-1.546 0.2955 1.803]  I1=[0.4986 61.4 49.04;377 377 377;-1.437 0.3077 1.863]  I2=[0.7398 68.64 54.28;377 377 377;-1.619 0.2843 1.749]  nHarmo=1  Measurements=None
      settings: SourceProductName=Simscape Power Systems
  836-862 301 : powerlib/Elements/Distributed Parameters Line  Phases=3  Frequency=60  Resistance=R_301  Inductance=L_301  Capacitance=C_301  Length=280*ft2km  x1=[287.744791807787 23220.7079462666 23346.2225579366;376.991118430775 376.991118430775 376.991118430775;-1.40218228535806 0.250543541085646 1.80349310786819]  x2=[287.454930429706 23220.5766114251 23346.1106507684;376.991118430775 376.991118430775 376.991118430775;-1.40177733396922 0.250538661376674 1.80349779683638]  x3=[1.63435739867086 65.910644062533 56.2281823333814;376.991118430775 376.991118430775 376.991118430775;0.352832464196579 0.242964263201215 1.82969416194889]  x4=[1.85507816266078 69.292265369895 57.1455273057619;376.991118430775 376.991118430775 376.991118430775;-2.44946330133344 0.25763242146948 1.77760155941479]  x5=3.86117260974383e-07  V1=[565 2.234e+04 2.126e+04;377 377 377;-1.545 0.2958 1.803]  V2=[564.7 2.234e+04 2.125e+04;377 377 377;-1.545 0.2958 1.803]  I1=[1.465 63.39 51.16;377 377 377;0.1615 0.2892 1.831]  I2=[2.039 66.7 52.06;377 377 377;-2.338 0.3019 1.776]  nHarmo=1  Measurements=None
      settings: SourceProductName=Simscape Power Systems
  838 : Subsystem
  838 Y PQ : powerlib/Elements/Series RLC Load  LConnTagsString=a  RConnTagsString=__new0  NominalVoltage=1.0*14376.02  NominalFrequency=60  ActivePower="28e3/2  *a"  InductivePower=14e3/2*a  CapacitivePower=0  Setx0=off  InitialVoltage=0  SetiL0=off  InitialCurrent=0  Measurements=None  LoadType=constant PQ
      settings: SourceProductName=Simscape Electrical
  840 : powerlib/Measurements/Three-Phase V-I Measurement  VoltageMeasurement=phase-to-ground  SetLabelV=on  LabelV=V840  Vpu=off  VpuLL=off  CurrentMeasurement=yes  SetLabelI=on  LabelI=I840  Ipu=off  Pbase=100e6  Vbase=24900  OutputType=Complex  PhasorSimulation=on  PSBequivalent=0
      settings: SourceProductName=Simscape Electrical
  840 D I : powerlib/Elements/Three-Phase Series RLC Load  LConnTagsString=A|B|C  Configuration=Delta  NominalVoltage=1000  Vabc=[1e3 1e3 1e3]  Vabcp=[ 1.0 1.0 1.0]*24900  NominalFrequency=60  UnbalancedPower=on  ActivePower=10e3  InductivePower=100  CapacitivePower=100  Pabc=[10e3 9e3 11e3]  QLabc=[100 90 110]  QCabc=[100 90 110]  Pabcp=[18 22 1e-3 ]*1e3/2 *a  QLabcp=[9 11 0]*1e3/2 *a  QCabcp=[0 0 0]  Measurements=None  LoadType=constant I
      settings: SourceProductName=Simscape Electrical
  840 Y I : powerlib/Elements/Three-Phase Series RLC Load  LConnTagsString=A|B|C  Configuration=Y (grounded)  NominalVoltage=[ 1.0 1.0 1.0]*2401.78  Vabc=[ 1.0 1.0 1.0]*14376.02  Vabcp=[1e3 1e3 1e3]  NominalFrequency=60  UnbalancedPower=on  ActivePower=[9 9 9]*1e3  InductivePower=[7 7 7]*1e3  CapacitivePower=0  Pabc=[9 9 9]*1e3 *a  QLabc=[7 7 7]*1e3*a  QCabc=[0 0 0]  Pabcp=[10e3 9e3 11e3]  QLabcp=[100 90 110]  QCabcp=[100 90 110]  Measurements=None  LoadType=constant I
      settings: SourceProductName=Simscape Electrical
  842 : powerlib/Measurements/Three-Phase V-I Measurement  VoltageMeasurement=phase-to-ground  SetLabelV=on  LabelV=V842  Vpu=off  VpuLL=off  CurrentMeasurement=yes  SetLabelI=on  LabelI=I842  Ipu=off  Pbase=100e6  Vbase=24900  OutputType=Complex  PhasorSimulation=on  PSBequivalent=0
      settings: SourceProductName=Simscape Electrical
  842 Y PQ : powerlib/Elements/Three-Phase Series RLC Load  LConnTagsString=A|B|C  Configuration=Y (grounded)  NominalVoltage=1000  Vabc=[ 1.0 1.0 1.0]*14376.02  Vabcp=[1e3 1e3 1e3]  NominalFrequency=60  UnbalancedPower=on  ActivePower=10e3  InductivePower=100  CapacitivePower=100  Pabc="[9 1e-3  1e-3 ]*1e3/2 *a"  QLabc=[5 0 0]*1e3/2 *a  QCabc=[0 0 0]  Pabcp=[10e3 9e3 11e3]  QLabcp=[100 90 110]  QCabcp=[100 90 110]  Measurements=None  LoadType=constant PQ
      settings: SourceProductName=Simscape Electrical
  842-844 301 : powerlib/Elements/Distributed Parameters Line  Phases=3  Frequency=60  Resistance=R_301  Inductance=L_301  Capacitance=C_301  Length=1350*ft2km  x1=[292.992794774887 23235.0415061901 23359.9419144581;376.991118430775 376.991118430775 376.991118430775;-1.40632937418497 0.249978913362739 1.80290889352913]  x2=[291.397612234942 23229.1212453125 23353.9940891929;376.991118430775 376.991118430775 376.991118430775;-1.40365053032829 0.249529691873541 1.8024910118817]  x3=[1.96050032599302 49.4264529989371 38.3187515496704;376.991118430775 376.991118430775 376.991118430775;0.299411848764399 -0.0554147756719583 1.48957050335778]  x4=[2.14111753181389 89.259531279842 77.7581729929231;376.991118430775 376.991118430775 376.991118430775;-2.54249541332221 0.41646553605603 1.95467291724073]  x5=1.86163679398363e-06  V1=[570.8 2.237e+04 2.128e+04;377 377 377;-1.544 0.2951 1.803]  V2=[568.6 2.236e+04 2.127e+04;377 377 377;-1.543 0.295 1.803]  I1=[2.263 41.11 29.63;377 377 377;0.3794 0.362 1.994]  I2=[2.934 89.17 74.35;377 377 377;-2.353 0.2638 1.727]  nHarmo=1  Measurements=None
      settings: SourceProductName=Simscape Power Systems
  844 : powerlib/Measurements/Three-Phase V-I Measurement  VoltageMeasurement=phase-to-ground  SetLabelV=on  LabelV=V844  Vpu=off  VpuLL=off  CurrentMeasurement=yes  SetLabelI=on  LabelI=I844  Ipu=off  Pbase=100e6  Vbase=24900  OutputType=Complex  PhasorSimulation=on  PSBequivalent=0
      settings: SourceProductName=Simscape Electrical
  844 Y PQ : powerlib/Elements/Three-Phase Series RLC Load  LConnTagsString=A|B|C  Configuration=Y (grounded)  NominalVoltage=1000  Vabc=[ 1.0 1.0 1.0]*14376.02  Vabcp=[1e3 1e3 1e3]  NominalFrequency=60  UnbalancedPower=on  ActivePower=10e3  InductivePower=100  CapacitivePower=100  Pabc="[9 1e-3  1e-3 ]*1e3/2 *a"  QLabc=[5 0 0]*1e3/2 *a  QCabc=[0 0 0]  Pabcp=[10e3 9e3 11e3]  QLabcp=[100 90 110]  QCabcp=[100 90 110]  Measurements=None  LoadType=constant PQ
      settings: SourceProductName=Simscape Electrical
  844 Y PQ1 : powerlib/Elements/Three-Phase Series RLC Load  LConnTagsString=A|B|C  Configuration=Y (grounded)  NominalVoltage=1000  Vabc=[ 1.0 1.0 1.0]*14376.02  Vabcp=[1e3 1e3 1e3]  NominalFrequency=60  UnbalancedPower=on  ActivePower=10e3  InductivePower=100  CapacitivePower=100  Pabc="[1e-3  25 20]*1e3/2 *a"  QLabc=[0 12 11]*1e3/2*a  QCabc=[0 0 0]  Pabcp=[10e3 9e3 11e3]  QLabcp=[100 90 110]  QCabcp=[100 90 110]  Measurements=None  LoadType=constant PQ
      settings: SourceProductName=Simscape Electrical
  844 Y Z : powerlib/Elements/Three-Phase Series RLC Load  LConnTagsString=A|B|C  Configuration=Y (grounded)  NominalVoltage=[ 1.0 1.0 1.0]*2401.78  Vabc=[ 1.0 1.0 1.0]*14376.02  Vabcp=[1e3 1e3 1e3]  NominalFrequency=60  UnbalancedPower=on  ActivePower=[135 135 135]*1e3  InductivePower=[105 105 105]*1e3  CapacitivePower=0  Pabc=[135 135 135]*1e3 *a  QLabc=[105 105 105]*1e3*a  QCabc=[0 0 0]  Pabcp=[10e3 9e3 11e3]  QLabcp=[100 90 110]  QCabcp=[100 90 110]  Measurements=None  LoadType=constant Z
      settings: SourceProductName=Simscape Electrical
  844 Yg Z : powerlib/Elements/Three-Phase Series RLC Load  LConnTagsString=A|B|C  Configuration=Y (grounded)  NominalVoltage=1000  Vabc=[ 1.0 1.0 1.0]*14376.02  Vabcp=[1e3 1e3 1e3]  NominalFrequency=60  UnbalancedPower=on  ActivePower=0  InductivePower=0  CapacitivePower=100  Pabc=[0 0 0]  QLabc=[0 0 0]  QCabc=[100 100 100]*1e3*a  Pabcp=[10e3 9e3 11e3]  QLabcp=[100 90 110]  QCabcp=[100 90 110]  Measurements=None  LoadType=constant Z
      settings: SourceProductName=Simscape Electrical
  844-846 301 : powerlib/Elements/Distributed Parameters Line  Phases=3  Frequency=60  Resistance=R_301  Inductance=L_301  Capacitance=C_301  Length=3640*ft2km  x1=[291.397612234942 23229.1212453125 23353.9940891929;376.991118430775 376.991118430775 376.991118430775;-1.404841025906 0.248559455400489 1.80153599035327]  x2=[288.186782571765 23232.3273075041 23357.9148969038;376.991118430775 376.991118430775 376.991118430775;-1.3981604343581 0.247681089535611 1.80078236470264]  x3=[1.55233931836138 65.0387016031467 54.4696064041663;376.991118430775 376.991118430775 376.991118430775;0.171681626208045 0.00668082369064243 1.5566497750656]  x4=[1.6780383231241 73.4315931945033 61.7191174133511;376.991118430775 376.991118430775 376.991118430775;-2.58372912014877 0.460057535478458 2.01503905929807]  x5=5.01952439266698e-06  V1=[568.6 2.236e+04 2.127e+04;377 377 377;-1.544 0.294 1.802]  V2=[564.5 2.236e+04 2.126e+04;377 377 377;-1.543 0.2936 1.802]  I1=[1.562 56.53 44.01;377 377 377;0.1954 0.2343 1.783]  I2=[2.149 73.53 59.05;377 377 377;-2.343 0.3382 1.815]  nHarmo=1  Measurements=None
      settings: SourceProductName=Simscape Power Systems
  846 : powerlib/Measurements/Three-Phase V-I Measurement  VoltageMeasurement=phase-to-ground  SetLabelV=on  LabelV=V846  Vpu=off  VpuLL=off  CurrentMeasurement=yes  SetLabelI=on  LabelI=I846  Ipu=off  Pbase=100e6  Vbase=24900  OutputType=Complex  PhasorSimulation=on  PSBequivalent=0
      settings: SourceProductName=Simscape Electrical
  846 Y PQ : powerlib/Elements/Three-Phase Series RLC Load  LConnTagsString=A|B|C  Configuration=Y (grounded)  NominalVoltage=1000  Vabc=[ 1.0 1.0 1.0]*14376.02  Vabcp=[1e3 1e3 1e3]  NominalFrequency=60  UnbalancedPower=on  ActivePower=10e3  InductivePower=100  CapacitivePower=100  Pabc="[1e-3  25 20]*1e3/2 *a"  QLabc=[0 12 11]*1e3/2*a  QCabc=[0 0 0]  Pabcp=[10e3 9e3 11e3]  QLabcp=[100 90 110]  QCabcp=[100 90 110]  Measurements=None  LoadType=constant PQ
      settings: SourceProductName=Simscape Electrical
  846 Y PQ1 : powerlib/Elements/Three-Phase Series RLC Load  LConnTagsString=A|B|C  Configuration=Y (grounded)  NominalVoltage=1000  Vabc=[ 1.0 1.0 1.0]*14376.02  Vabcp=[1e3 1e3 1e3]  NominalFrequency=60  UnbalancedPower=on  ActivePower=10e3  InductivePower=100  CapacitivePower=100  Pabc="[1e-3  23 1e-3 ]*1e3/2 *a"  QLabc=[0 11 0]*1e3/2 *a  QCabc=[0 0 0]  Pabcp=[10e3 9e3 11e3]  QLabcp=[100 90 110]  QCabcp=[100 90 110]  Measurements=None  LoadType=constant PQ
      settings: SourceProductName=Simscape Electrical
  846-848 301 : powerlib/Elements/Distributed Parameters Line  Phases=3  Frequency=60  Resistance=R_301  Inductance=L_301  Capacitance=C_301  Length=530*ft2km  x1=[288.186782571765 23232.3273075041 23357.9148969038;376.991118430775 376.991118430775 376.991118430775;-1.3965436477875 0.248998746929145 1.80207935900545]  x2=[288.025906264868 23233.0118818752 23358.8274840397;376.991118430775 376.991118430775 376.991118430775;-1.39663991886419 0.2488775181081 1.80196391137772]  x3=[0.295283708861168 66.4895165315263 56.1372820397785;376.991118430775 376.991118430775 376.991118430775;0.387033055300694 0.0170105189787141 1.53810300783125]  x4=[0.749300498835152 72.1698485679744 60.9663722227776;376.991118430775 376.991118430775 376.991118430775;-1.79212831686771 0.462100978986082 2.04438442512839]  x5=7.30864815415796e-07  V1=[564.5 2.236e+04 2.126e+04;377 377 377;-1.541 0.2949 1.803]  V2=[564.2 2.235e+04 2.126e+04;377 377 377;-1.541 0.2949 1.803]  I1=[0.3256 57.99 45.26;377 377 377;0.3373 0.2412 1.754]  I2=[1.367 72.3 58.04;377 377 377;-1.77 0.3378 1.841]  nHarmo=1  Measurements=None
      settings: SourceProductName=Simscape Power Systems
  "848 " : powerlib/Measurements/Three-Phase V-I Measurement  VoltageMeasurement=phase-to-ground  SetLabelV=on  LabelV=V848  Vpu=off  VpuLL=off  CurrentMeasurement=yes  SetLabelI=on  LabelI=I848  Ipu=off  Pbase=100e6  Vbase=24900  OutputType=Complex  PhasorSimulation=on  PSBequivalent=0
      settings: SourceProductName=Simscape Electrical
  848 D PQ : powerlib/Elements/Three-Phase Series RLC Load  LConnTagsString=A|B|C  Configuration=Delta  NominalVoltage=1000  Vabc=[ 1.0 1.0 1.0]*14376.02  Vabcp=[ 1.0 1.0 1.0]*24900  NominalFrequency=60  UnbalancedPower=on  ActivePower=10e3  InductivePower=100  CapacitivePower=100  Pabc=[20 20 20]*1e3  QLabc=[16 16 16]*1e3  QCabc=[0 0 0]  Pabcp=[20 20 20]*1e3 *a  QLabcp=[16 16 16]*1e3 *a  QCabcp=[0 0 0]  Measurements=None  LoadType=constant PQ
      settings: SourceProductName=Simscape Electrical
  848 Y PQ : powerlib/Elements/Three-Phase Series RLC Load  LConnTagsString=A|B|C  Configuration=Y (grounded)  NominalVoltage=1000  Vabc=[ 1.0 1.0 1.0]*14376.02  Vabcp=[1e3 1e3 1e3]  NominalFrequency=60  UnbalancedPower=on  ActivePower=10e3  InductivePower=100  CapacitivePower=100  Pabc="[1e-3  23 1e-3 ]*1e3/2 *a"  QLabc=[0 11 0]*1e3/2 *a  QCabc=[0 0 0]  Pabcp=[10e3 9e3 11e3]  QLabcp=[100 90 110]  QCabcp=[100 90 110]  Measurements=None  LoadType=constant PQ
      settings: SourceProductName=Simscape Electrical
  848 Y Z : powerlib/Elements/Three-Phase Series RLC Load  LConnTagsString=A|B|C  Configuration=Y (grounded)  NominalVoltage=1000  Vabc=[ 1.0 1.0 1.0]*14376.02  Vabcp=[1e3 1e3 1e3]  NominalFrequency=60  UnbalancedPower=on  ActivePower=0  InductivePower=0  CapacitivePower=100  Pabc=[0 0 0]  QLabc=[0 0 0]  QCabc=[150 150 150]*1e3*a  Pabcp=[10e3 9e3 11e3]  QLabcp=[100 90 110]  QCabcp=[100 90 110]  Measurements=None  LoadType=constant Z
      settings: SourceProductName=Simscape Electrical
  850 : powerlib/Measurements/Three-Phase V-I Measurement  VoltageMeasurement=phase-to-ground  SetLabelV=on  LabelV=V850  Vpu=off  VpuLL=off  CurrentMeasurement=no  SetLabelI=off  LabelI=I815  Ipu=off  Pbase=100e6  Vbase=24900  OutputType=Complex  PhasorSimulation=on  PSBequivalent=0
      settings: SourceProductName=Simscape Electrical
  850-816 301 : powerlib/Elements/Distributed Parameters Line  Phases=3  Frequency=60  Resistance=R_301  Inductance=L_301  Capacitance=C_301  Length=310*ft2km  x1=[541.683717853495 24529.4812379324 24692.3879781101;376.991118430775 376.991118430775 376.991118430775;-1.38212043330038 0.270283914431195 1.83090135438667]  x2=[540.68108300544 24522.5116299881 24686.5051711599;376.991118430775 376.991118430775 376.991118430775;-1.38584501691876 0.270219310828447 1.8307843749951]  x3=[10.6286670924887 15.05593829161 2.7236431303072;376.991118430775 376.991118430775 376.991118430775;2.05820520906254 1.34433579962729 2.80976828238014]  x4=[11.762613008365 136.267133379653 118.356374533044;376.991118430775 376.991118430775 376.991118430775;-1.11314657098672 0.172892726111623 1.81167843127001]  x5=4.27486967507352e-07  V1=[322.1 2.375e+04 2.363e+04;377 377 377;-1.555 0.2745 1.834]  V2=[320.6 2.373e+04 2.361e+04;377 377 377;-1.566 0.2746 1.834]  I1=[17.89 80.08 64.4;377 377 377;1.9 2.507 -1.985]  I2=[18.56 197.8 169.7;377 377 377;-1.254 -0.05064 1.594]  nHarmo=1  Measurements=None
      settings: SourceProductName=Simscape Power Systems
  "852 " : powerlib/Measurements/Three-Phase V-I Measurement  VoltageMeasurement=phase-to-ground  SetLabelV=on  LabelV=V852  Vpu=off  VpuLL=off  CurrentMeasurement=no  SetLabelI=off  LabelI=I815  Ipu=off  Pbase=100e6  Vbase=24900  OutputType=Complex  PhasorSimulation=on  PSBequivalent=0
      settings: SourceProductName=Simscape Electrical
  852-832 301 : powerlib/Elements/Distributed Parameters Line  Phases=3  Frequency=60  Resistance=R_301  Inductance=L_301  Capacitance=C_301  Length=10*ft2km  x1=[320.510745324123 23350.0826623343 23477.2066742434;376.991118430775 376.991118430775 376.991118430775;-1.41642294325164 0.253510157241638 1.80733264625147]  x2=[320.48155576948 23349.9161493877 23477.0352904044;376.991118430775 376.991118430775 376.991118430775;-1.41642869803416 0.253507738297541 1.80732918749187]  x3=[4.26253081481009 18.8846705679913 5.37929829471012;376.991118430775 376.991118430775 376.991118430775;0.90743627531155 0.520507002264654 2.34547494735552]  x4=[4.76862099934502 117.867925628924 109.404567602357;376.991118430775 376.991118430775 376.991118430775;-2.12686217426524 0.211222217554339 1.78212490717883]  x5=1.37899021776565e-08  V1=[606.1 2.261e+04 2.152e+04;377 377 377;-1.525 0.2949 1.807]  V2=[606 2.261e+04 2.152e+04;377 377 377;-1.525 0.2949 1.807]  I1=[6.407 59.01 56.95;377 377 377;1.236 2.33 -2.02]  I2=[7.652 166.7 152.9;377 377 377;-1.841 -0.02726 1.569]  nHarmo=1  Measurements=None
      settings: SourceProductName=Simscape Power Systems
  854 : powerlib/Measurements/Three-Phase V-I Measurement  VoltageMeasurement=phase-to-ground  SetLabelV=on  LabelV=V854  Vpu=off  VpuLL=off  CurrentMeasurement=yes  SetLabelI=on  LabelI=I854  Ipu=off  Pbase=100e6  Vbase=24900  OutputType=Complex  PhasorSimulation=on  PSBequivalent=0
      settings: SourceProductName=Simscape Electrical
  854 Y PQ : powerlib/Elements/Series RLC Load  LConnTagsString=a  RConnTagsString=__new0  NominalVoltage=1.0*14376.02  NominalFrequency=60  ActivePower=4e3/2 *a  InductivePower=2e3/2*a  CapacitivePower=0  Setx0=off  InitialVoltage=0  SetiL0=off  InitialCurrent=0  Measurements=None  LoadType=constant PQ
      settings: SourceProductName=Simscape Electrical
  854-852 301 : powerlib/Elements/Distributed Parameters Line  Phases=3  Frequency=60  Resistance=R_301  Inductance=L_301  Capacitance=C_301  Length=36830*ft2km  x1=[428.013916342019 23961.6924006652 24107.7905484182;376.991118430775 376.991118430775 376.991118430775;-1.4195257125668 0.246860171897156 1.8046035463029]  x2=[320.510750551727 23350.0827618512 23477.2067782518;376.991118430775 376.991118430775 376.991118430775;-1.43556446764361 0.237910110107005 1.79197723438184]  x3=[4.14771184039044 19.5649017813372 6.19060942614752;376.991118430775 376.991118430775 376.991118430775;0.868350068756522 0.467351915373496 2.21954230129409]  x4=[4.72586642131339 115.319030647634 107.486909595551;376.991118430775 376.991118430775 376.991118430775;-2.14612489700452 0.195426749046015 1.76668552111045]  x5=5.0788209720309e-05  V1=[194.3 2.238e+04 2.233e+04;377 377 377;-2.51 0.2624 1.812]  V2=[335.9 2.09e+04 2.093e+04;377 377 377;2.838 0.2667 1.805]  I1=[11.06 63.46 58.4;377 377 377;1.41 2.436 -2.064]  I2=[11.17 167.4 151.6;377 377 377;-1.777 -0.05959 1.543]  nHarmo=1  Measurements=None
      settings: SourceProductName=Simscape Power Systems
  854-856 303 : powerlib/Elements/Distributed Parameters Line  Phases=1  Frequency=60  Resistance=R_303(2,2)  Inductance=L_303(2,2)  Capacitance=C_303(2,2)  Length=23330*ft2km  x1=[19878.1425167525;376.991118430775;-2.16269607865136]  x2=[19876.3496970908;376.991118430775;-2.16281520406748]  x3=[32.81492276286;376.991118430775;-2.17098632006957]  x4=[33.1916816202015;376.991118430775;-2.16568268529717]  x5=2.9363349960162e-05  V1=[1.851e+04;377;-2.166]  V2=[1.851e+04;377;-2.166]  I1=[30.56;377;-2.174]  I2=[30.91;377;-2.169]  nHarmo=1  Measurements=None
      settings: SourceProductName=Simscape Power Systems
  856 : Subsystem
  856 Y PQ : powerlib/Elements/Series RLC Load  LConnTagsString=a  RConnTagsString=__new0  NominalVoltage=1.0*14376.02  NominalFrequency=60  ActivePower=4e3/2*a  InductivePower=2e3/2*a  CapacitivePower=0  Setx0=off  InitialVoltage=0  SetiL0=off  InitialCurrent=0  Measurements=None  LoadType=constant PQ
      settings: SourceProductName=Simscape Electrical
  858 : powerlib/Measurements/Three-Phase V-I Measurement  VoltageMeasurement=phase-to-ground  SetLabelV=on  LabelV=V858  Vpu=off  VpuLL=off  CurrentMeasurement=yes  SetLabelI=on  LabelI=I858  Ipu=off  Pbase=100e6  Vbase=24900  OutputType=Complex  PhasorSimulation=on  PSBequivalent=0
      settings: SourceProductName=Simscape Electrical
  858 D PQ : powerlib/Elements/Three-Phase Series RLC Load  LConnTagsString=A|B|C  Configuration=Delta  NominalVoltage=1000  Vabc=[1e3 1e3 1e3]  Vabcp=[ 1.0 1.0 1.0]*24900  NominalFrequency=60  UnbalancedPower=on  ActivePower=10e3  InductivePower=100  CapacitivePower=100  Pabc=[10e3 9e3 11e3]  QLabc=[100 90 110]  QCabc=[100 90 110]  Pabcp=[4 15 13]*1e3/2 *a  QLabcp=[2 8 7]*1e3/2 *a  QCabcp=[0 0 0]  Measurements=None  LoadType=constant PQ
      settings: SourceProductName=Simscape Electrical
  858 D Z : powerlib/Elements/Three-Phase Series RLC Load  LConnTagsString=A|B|C  Configuration=Delta  NominalVoltage=1000  Vabc=[1e3 1e3 1e3]  Vabcp=[ 1.0 1.0 1.0]*24900  NominalFrequency=60  UnbalancedPower=on  ActivePower=10e3  InductivePower=100  CapacitivePower=100  Pabc=[10e3 9e3 11e3]  QLabc=[100 90 110]  QCabc=[100 90 110]  Pabcp=[7 2 6]*1e3/2 *a  QLabcp=[3 1 3]*1e3/2 *a  QCabcp=[0 0 0]  Measurements=None  LoadType=constant Z
      settings: SourceProductName=Simscape Electrical
  858 Y PQ : powerlib/Elements/Series RLC Load  LConnTagsString=a  RConnTagsString=__new0  NominalVoltage=1.0*14376.02  NominalFrequency=60  ActivePower="2e3/2  *a"  InductivePower=1e3/2*a  CapacitivePower=0  Setx0=off  InitialVoltage=0  SetiL0=off  InitialCurrent=0  Measurements=None  LoadType=constant PQ
      settings: SourceProductName=Simscape Electrical
  858-834 301 : powerlib/Elements/Distributed Parameters Line  Phases=3  Frequency=60  Resistance=R_301  Inductance=L_301  Capacitance=C_301  Length=5830*ft2km  x1=[308.059778746511 23297.1351077948 23423.0500557617;376.991118430775 376.991118430775 376.991118430775;-1.41580390797501 0.249736039788633 1.80317224463582]  x2=[293.318135105792 23236.3015016255 23361.1779978373;376.991118430775 376.991118430775 376.991118430775;-1.40903661722633 0.248173499272881 1.80112769326623]  x3=[3.74630437705133 33.5120412319393 21.0285111419158;376.991118430775 376.991118430775 376.991118430775;0.694544265710225 0.132891240970656 1.51195659423647]  x4=[4.12057373613207 101.724532948113 93.2300896021391;376.991118430775 376.991118430775 376.991118430775;-2.3100370257412 0.285473748050575 1.86525557936381]  x5=8.03951296957375e-06  V1=[590 2.25e+04 2.141e+04;377 377 377;-1.537 0.2928 1.803]  V2=[571.2 2.238e+04 2.128e+04;377 377 377;-1.546 0.2933 1.801]  I1=[4.637 31.64 16;377 377 377;0.9907 1.498 -2.371]  I2=[5.722 122.5 112.4;377 377 377;-2.024 0.0481 1.678]  nHarmo=1  Measurements=None
      settings: SourceProductName=Simscape Power Systems
  858-864 1 : powerlib/Elements/Distributed Parameters Line  Phases=1  Frequency=60  Resistance=R_302(1,1)  Inductance=L_302(1,1)  Capacitance=C_302(1,1)  Length=1620*ft2km  x1=[18554.7555233539;376.991118430775;-0.0393722029480391]  x2=[18554.6634301541;376.991118430775;-0.0393728869880166]  x3=[31.1686102491296;376.991118430775;-0.038704179860409]  x4=[31.347908623906;376.991118430775;-0.0408038314108909]  x5=2.03894671819385e-06  V1=[1.763e+04;377;0.005038]  V2=[1.763e+04;377;0.005037]  I1=[29.61;377;0.005706]  I2=[29.78;377;0.003606]  nHarmo=1  Measurements=None
      settings: SourceProductName=Simscape Power Systems
  860 : powerlib/Measurements/Three-Phase V-I Measurement  VoltageMeasurement=phase-to-ground  SetLabelV=on  LabelV=V860  Vpu=off  VpuLL=off  CurrentMeasurement=no  SetLabelI=on  LabelI=I860  Ipu=off  Pbase=100e6  Vbase=24900  OutputType=Complex  PhasorSimulation=on  PSBequivalent=0
      settings: SourceProductName=Simscape Electrical
  860 D PQ : powerlib/Elements/Three-Phase Series RLC Load  LConnTagsString=A|B|C  Configuration=Delta  NominalVoltage=1000  Vabc=[ 1.0 1.0 1.0]*14376.02  Vabcp=[ 1.0 1.0 1.0]*24900  NominalFrequency=60  UnbalancedPower=on  ActivePower=10e3  InductivePower=100  CapacitivePower=100  Pabc=[30 10 42]*1e3/2  QLabc=[15 6 22]*1e3/2  QCabc=[0 0 0]  Pabcp=[30 10 42]*1e3/2 *a  QLabcp=[15 6 22]*1e3/2 *a  QCabcp=[0 0 0]  Measurements=None  LoadType=constant PQ
      settings: SourceProductName=Simscape Electrical
  860 D Z : powerlib/Elements/Three-Phase Series RLC Load  LConnTagsString=A|B|C  Configuration=Delta  NominalVoltage=1000  Vabc=[1e3 1e3 1e3]  Vabcp=[ 1.0 1.0 1.0]*24900  NominalFrequency=60  UnbalancedPower=on  ActivePower=10e3  InductivePower=100  CapacitivePower=100  Pabc=[10e3 9e3 11e3]  QLabc=[100 90 110]  QCabc=[100 90 110]  Pabcp=[16 20 110]*1e3/2 *a  QLabcp=[8 10 55]*1e3/2*a  QCabcp=[0 0 0]  Measurements=None  LoadType=constant Z
      settings: SourceProductName=Simscape Electrical
  860 Y PQ : powerlib/Elements/Three-Phase Series RLC Load  LConnTagsString=A|B|C  Configuration=Y (grounded)  NominalVoltage=[ 1.0 1.0 1.0]*2401.78  Vabc=[ 1.0 1.0 1.0]*14376.02  Vabcp=[1e3 1e3 1e3]  NominalFrequency=60  UnbalancedPower=on  ActivePower=[20 20 20]*1e3  InductivePower=[16 16 16]*1e3  CapacitivePower=0  Pabc="[20 20 20]*1e3  *a"  QLabc=[16 16 16]*1e3*a  QCabc=[0 0 0]  Pabcp=[10e3 9e3 11e3]  QLabcp=[100 90 110]  QCabcp=[100 90 110]  Measurements=None  LoadType=constant PQ
      settings: SourceProductName=Simscape Electrical
  860-836 301 : powerlib/Elements/Distributed Parameters Line  Phases=3  Frequency=60  Resistance=R_301  Inductance=L_301  Capacitance=C_301  Length=2680*ft2km  x1=[290.754060428224 23226.5580690742 23351.6426236293;376.991118430775 376.991118430775 376.991118430775;-1.40654391474606 0.249572685573063 1.80242726067505]  x2=[287.744791807787 23220.7079462666 23346.2225579366;376.991118430775 376.991118430775 376.991118430775;-1.40342996631287 0.249526699367164 1.80249221194319]  x3=[1.6896897054132 61.4071857054045 52.5804926002064;376.991118430775 376.991118430775 376.991118430775;0.452434491122907 0.273979785517735 1.87854297727353]  x4=[1.96410180336821 73.6181673132931 60.8983147229754;376.991118430775 376.991118430775 376.991118430775;-2.3759257020233 0.22813051062361 1.73574298898723]  x5=3.69569378361195e-06  V1=[568.3 2.236e+04 2.127e+04;377 377 377;-1.547 0.2948 1.802]  V2=[565 2.234e+04 2.126e+04;377 377 377;-1.547 0.2947 1.802]  I1=[1.543 52.64 43.37;377 377 377;0.4547 0.373 1.967]  I2=[2.346 77.55 60.71;377 377 377;-2.188 0.2407 1.684]  nHarmo=1  Measurements=None
      settings: SourceProductName=Simscape Power Systems
  862 : powerlib/Measurements/Three-Phase V-I Measurement  VoltageMeasurement=phase-to-ground  SetLabelV=on  LabelV=V862  Vpu=off  VpuLL=off  CurrentMeasurement=yes  SetLabelI=on  LabelI=I862  Ipu=off  Pbase=100e6  Vbase=24900  OutputType=Complex  PhasorSimulation=on  PSBequivalent=0
      settings: SourceProductName=Simscape Electrical
  862 Y PQ : powerlib/Elements/Series RLC Load  LConnTagsString=a  RConnTagsString=__new0  NominalVoltage=1.0*14376.02  NominalFrequency=60  ActivePower="28e3/2  *a"  InductivePower=14e3/2*a  CapacitivePower=0  Setx0=off  InitialVoltage=0  SetiL0=off  InitialCurrent=0  Measurements=None  LoadType=constant PQ
      settings: SourceProductName=Simscape Electrical
  862-838 304 : powerlib/Elements/Distributed Parameters Line  Phases=1  Frequency=60  Resistance=R_304(2,2)  Inductance=L_304(2,2)  Capacitance=C_304(2,2)  Length=4860*ft2km  x1=[19242.9311895757;376.991118430775;-2.17068944421983]  x2=[19239.8238859855;376.991118430775;-2.17072169556122]  x3=[32.344238524956;376.991118430775;-2.15295649377938]  x4=[34.9423675887561;376.991118430775;-2.18934348983144]  x5=6.08033278760362e-06  V1=[1.863e+04;377;-2.167]  V2=[1.863e+04;377;-2.167]  I1=[31.32;377;-2.149]  I2=[33.83;377;-2.185]  nHarmo=1  Measurements=None
      settings: SourceProductName=Simscape Power Systems
  864 : Subsystem
  864 Y PQ : powerlib/Elements/Series RLC Load  LConnTagsString=a  RConnTagsString=__new0  NominalVoltage=1.0*14376.02  NominalFrequency=60  ActivePower=2e3/2 *a  InductivePower=1e3/2*a  CapacitivePower=0  Setx0=off  InitialVoltage=0  SetiL0=off  InitialCurrent=0  Measurements=None  LoadType=constant PQ
      settings: SourceProductName=Simscape Electrical
  888 : powerlib/Measurements/Three-Phase V-I Measurement  VoltageMeasurement=phase-to-ground  SetLabelV=on  LabelV=V888  Vpu=off  VpuLL=off  CurrentMeasurement=yes  SetLabelI=on  LabelI=I888  Ipu=off  Pbase=100e6  Vbase=24900  OutputType=Complex  PhasorSimulation=on  PSBequivalent=0
      settings: SourceProductName=Simscape Electrical
  888-890 300 : powerlib/Elements/Distributed Parameters Line  Phases=3  Frequency=60  Resistance=R_300  Inductance=L_300  Capacitance=C_300  Length=10560*ft2km  x1=[99.6980242017348 3688.9813981404 3626.52541617421;376.991118430775 376.991118430775 376.991118430775;0.75488979279773 1.67900252779306 0.124685431963456]  x2=[113.337200137723 3421.56349508032 3351.33624588155;376.991118430775 376.991118430775 376.991118430775;0.650197576424144 1.66952431229999 0.1079228659742]  x3=[3.19049167091697 89.6329875412526 90.4532690093775;376.991118430775 376.991118430775 376.991118430775;-0.879739309393591 -1.99446814553166 2.74253328805009]  x4=[3.20220480820018 108.492438050678 105.877855430453;376.991118430775 376.991118430775 376.991118430775;2.18158048297168 1.2451937510369 -0.318643292040692]  x5=1.41710191462344e-05  V1=[204.8 3466 3295;377 377 377;2.308 0.231 1.747]  V2=[241.9 2808 2642;377 377 377;2.383 0.205 1.704]  I1=[7.634 235.1 225.3;377 377 377;1.85 2.866 -1.923]  I2=[7.165 251.7 238.3;377 377 377;-1.327 -0.2403 1.249]  nHarmo=1  Measurements=None
      settings: SourceProductName=Simscape Power Systems
  890 : powerlib/Measurements/Three-Phase V-I Measurement  VoltageMeasurement=phase-to-ground  SetLabelV=on  LabelV=V890  Vpu=off  VpuLL=off  CurrentMeasurement=yes  SetLabelI=on  LabelI=I890  Ipu=off  Pbase=100e6  Vbase=4160  OutputType=Complex  PhasorSimulation=on  PSBequivalent=0
      settings: SourceProductName=Simscape Electrical
  890 D I : powerlib/Elements/Three-Phase Series RLC Load  LConnTagsString=A|B|C  Configuration=Delta  NominalVoltage=1000  Vabc=[1e3 1e3 1e3]  Vabcp=[ 1.0 1.0 1.0]*4160  NominalFrequency=60  UnbalancedPower=on  ActivePower=10e3  InductivePower=100  CapacitivePower=100  Pabc=[10e3 9e3 11e3]  QLabc=[100 90 110]  QCabc=[100 90 110]  Pabcp=[150 150 150]*1e3 *a  QLabcp=[75 75 75]*1e3 *a  QCabcp=[0 0 0]  Measurements=None  LoadType=constant I
      settings: SourceProductName=Simscape Electrical
  Ground{1..14} (14 alike) : powerlib/Elements/Ground  LConnTagsString=a
      settings: SourceProductName=Simscape Electrical
  Node Voltages : Subsystem
  RG10 : powerlib/Measurements/Three-Phase V-I Measurement  VoltageMeasurement=phase-to-ground  SetLabelV=on  LabelV=RG10  Vpu=off  VpuLL=off  CurrentMeasurement=no  SetLabelI=off  LabelI=I815  Ipu=off  Pbase=100e6  Vbase=24900  OutputType=Complex  PhasorSimulation=on  PSBequivalent=0
      settings: SourceProductName=Simscape Electrical
  RG11 : powerlib/Measurements/Three-Phase V-I Measurement  VoltageMeasurement=phase-to-ground  SetLabelV=on  LabelV=RG11  Vpu=off  VpuLL=off  CurrentMeasurement=no  SetLabelI=off  LabelI=I815  Ipu=off  Pbase=100e6  Vbase=24900  OutputType=Complex  PhasorSimulation=on  PSBequivalent=0
      settings: SourceProductName=Simscape Electrical
  Regulator 1 : Subsystem
  Regulator 2 : Subsystem
  Regulator Taps : Subsystem
  Series RLC Branch3 : powerlib/Elements/Series RLC Branch  LConnTagsString=__new0  RConnTagsString=__new0  BranchType=R  Resistance=.001  Inductance=0  SetiL0=off  InitialCurrent=0  Capacitance=0  Setx0=off  InitialVoltage=0  Measurements=None
      settings: SourceProductName=Simscape Electrical
  Series RLC Branch4 : powerlib/Elements/Series RLC Branch  LConnTagsString=__new0  RConnTagsString=__new0  BranchType=R  Resistance=.001  Inductance=0  SetiL0=off  InitialCurrent=0  Capacitance=0  Setx0=off  InitialVoltage=0  Measurements=None
      settings: SourceProductName=Simscape Electrical
  Series RLC Branch5 : powerlib/Elements/Series RLC Branch  LConnTagsString=__new0  RConnTagsString=__new0  BranchType=R  Resistance=.001  Inductance=0  SetiL0=off  InitialCurrent=0  Capacitance=0  Setx0=off  InitialVoltage=0  Measurements=None
      settings: SourceProductName=Simscape Electrical
  Substation Power : Subsystem
  Three-Phase Transformer (Two Windings) : powerlib/Elements/Three-Phase Transformer (Two Windings)  Winding1Connection=Yg  Winding2Connection=Yg  CoreType=Three single-phase transformers  SetSaturation=off  Hysteresis=off  DataFile='hysteresis'  SetInitialFlux=off  Measurements=None  UNITS=pu  NominalPower=[ 500e3 , 60 ]  Winding1=[24900 0.019 0.0408]  Winding2=[4160 0.019 0.0408]  Rm=500  Lm=500  L0=0.5  Saturation=[ 0,0 ; 0.0024,1.2 ; 1.0,1.52 ]  InitialFluxes=[ 0.8 , -0.8 , 0.7 ]  BreakLoop=off  DiscreteSolver=Trapezoidal iterative  DataType=off  TransfoNumber=1
      settings: SourceProductName=Simscape Electrical
  Three-Phase Source : powerlib/Electrical Sources/Three-Phase Source  InternalConnection=Yg  VoltagePhases=on  Voltage=25e3  PhaseAngle=0  Voltage_phases=[ 1.05 1.05 1.05]*14376.02  PhaseAngles_phases=[ 0 -120 120]  Frequency=60  NonIdealSource=off  SpecifyImpedance=off  Resistance=1e-6  Inductance=1e-5  ShortCircuitLevel=100e6  BaseVoltage=24.9e3  XRratio=7  BusType=swing  Pref=10e3  Qref=0  Prefabc=[10e3, 10e3, 10e3]  Qrefabc=[0, 0, 0]  Qmin=-inf  Qmax=inf
      settings: SourceProductName=Simscape Electrical
  XF10 : powerlib/Measurements/Three-Phase V-I Measurement  VoltageMeasurement=phase-to-ground  SetLabelV=on  LabelV=XF10  Vpu=off  VpuLL=off  CurrentMeasurement=no  SetLabelI=on  LabelI=I888  Ipu=off  Pbase=100e6  Vbase=24900  OutputType=Complex  PhasorSimulation=on  PSBequivalent=0
      settings: SourceProductName=Simscape Electrical
  powergui : powerlib/powergui  Priority=1  SimulationMode=Phasor  SampleTime=Ts  frequency=60  Iterations=50  frequencyindice=60  Pbase=100e6  ErrMax=1e-4  UnitsV=kV  UnitsW=MW  buscounter=0  FunctionMessages=off  echomessages=on  EnableUseOfTLC=off  CurrentSourceSwitches=off  DisableSnubberDevices=off  DisableRonSwitches=off  DisableVfSwitches=off  DisplayEquations=off  AutomaticDiscreteSolvers=off  SolverType=Tustin  Interpol=off  ExternalGateDelay=off  methode=off  Ts=0  x0status=blocks  SPID=off  SwTol=0  HookPort=off  NonlinearTolerance=1e-4  nMaxIteration=100  ContinueOnMaxIteration=off  RestoreLinks=warning  ResistiveCurrentMeasurement=off  Frange=[0:2:500]  Ylog=off  Xlog=on  ShowGrid=off  save=off  variable=ZData  structure=0  ZoomFFT=off  StartTime=0.0  cycles=1  DisplayStyle=1  fundamental=60  FreqAxis=off  MaxFrequency=1000  frequencyindicesteady=1  RmsSteady=1  display=off
      settings: SourceProductName=Simscape Electrical
  tag scope: Reg1=global, Reg2=global
  wires:
  Regulator 2/1(Tap) -> [Reg2]
  Regulator 1/1(Tap) -> [Reg1]
  connections:
  838/LConn1 -- 838 Y PQ/LConn1
  862-838 304/RConn1 -- 838/RConn1
  856/LConn1 -- 856 Y PQ/LConn1
  854-856 303/RConn1 -- 856/RConn1
  864/LConn1 -- 864 Y PQ/LConn1
  858-864 1/RConn1 -- 864/RConn1
  826/LConn1 -- 826 Y I/LConn1
  826/RConn1 -- 824-826 303/RConn1
  822/LConn1 -- 822 Y PQ/LConn1
  820-822 302/RConn1 -- 822/RConn1
  820Y Z/LConn1 -- 818-820 302/RConn1 -- 820/RConn1
  816-818 302/RConn1 -- 818/RConn1
  810/LConn1 -- 810 Y I/LConn1
  808-810 303/RConn1 -- 810/RConn1
  Three-Phase Transformer (Two Windings)/RConn3 -- XF10/LConn3
  Three-Phase Transformer (Two Windings)/RConn2 -- XF10/LConn2
  Three-Phase Transformer (Two Windings)/RConn1 -- XF10/LConn1
  832 D Z/LConn2 -- 832-858 301/LConn2 -- 832/RConn2 -- Three-Phase Transformer (Two Windings)/LConn2
  832 D Z/LConn3 -- 832-858 301/LConn3 -- 832/RConn3 -- Three-Phase Transformer (Two Windings)/LConn1
  XF10/RConn3 -- 888/LConn3
  XF10/RConn2 -- 888/LConn2
  XF10/RConn1 -- 888/LConn1
  852-832 301/RConn3 -- 832/LConn3
  852-832 301/RConn2 -- 832/LConn2
  852-832 301/RConn1 -- 832/LConn1
  814-850 301/RConn3 -- 850/LConn3
  814-850 301/RConn2 -- 850/LConn2
  814-850 301/RConn1 -- 850/LConn1
  814-850 301/LConn3 -- RG10/RConn3
  814-850 301/LConn2 -- RG10/RConn2
  814-850 301/LConn1 -- RG10/RConn1
  812-814 300/RConn2 -- 814/LConn2
  812-814 300/RConn1 -- 814/LConn1
  812-814 300/RConn3 -- 814/LConn3
  852-832 301/LConn3 -- RG11/RConn3
  852-832 301/LConn2 -- RG11/RConn2
  852-832 301/LConn1 -- RG11/RConn1
  850-816 301/LConn1 -- 850/RConn1
  850-816 301/LConn2 -- 850/RConn2
  850-816 301/LConn3 -- 850/RConn3
  812-814 300/LConn3 -- 812/RConn3
  812-814 300/LConn2 -- 812/RConn2
  812-814 300/LConn1 -- 812/RConn1
  808-812 300/RConn3 -- 812/LConn3
  808-812 300/RConn2 -- 812/LConn2
  808-812 300/RConn1 -- 812/LConn1
  858 D Z/LConn2 -- 858-834 301/LConn2 -- 858 D PQ/LConn2 -- 858/RConn2
  858/RConn1 -- 858 D Z/LConn1 -- 858-864 1/LConn1 -- 858-834 301/LConn1 -- 858 D PQ/LConn1 -- 858 Y PQ/LConn1
  800/RConn3 -- Series RLC Branch5/LConn1
  800-802 300/LConn1 -- Series RLC Branch3/RConn1
  800/RConn2 -- Series RLC Branch4/LConn1
  800-802 300/LConn3 -- Series RLC Branch5/RConn1
  800-802 300/LConn2 -- Series RLC Branch4/RConn1
  800/RConn1 -- Series RLC Branch3/LConn1
  890/RConn1 -- 890 D I/LConn1
  890/RConn3 -- 890 D I/LConn3
  890/RConn2 -- 890 D I/LConn2
  832 D Z/LConn1 -- 832-858 301/LConn1 -- 832/RConn1 -- Three-Phase Transformer (Two Windings)/LConn3
  888-890 300/RConn2 -- 890/LConn2
  888-890 300/LConn3 -- 888/RConn3
  888-890 300/RConn1 -- 890/LConn1
  800/LConn2 -- Three-Phase Source/RConn2
  800/LConn3 -- Three-Phase Source/RConn3
  800/LConn1 -- Three-Phase Source/RConn1
  888-890 300/RConn3 -- 890/LConn3
  888-890 300/LConn2 -- 888/RConn2
  834-842 301/RConn2 -- 842/LConn2
  834-842 301/RConn1 -- 842/LConn1
  836-862 301/RConn3 -- 862/LConn3
  888-890 300/LConn1 -- 888/RConn1
  834-842 301/RConn3 -- 842/LConn3
  838 Y PQ/RConn1 -- Ground14/LConn1
  820Y Z/RConn1 -- Ground4/LConn1
  856 Y PQ/RConn1 -- Ground10/LConn1
  Ground9/LConn1 -- 854 Y PQ/RConn1
  836 D PQ/LConn1 -- 860-836 301/RConn1 -- 836/LConn1
  848 D PQ/LConn3 -- "848 "/RConn3 -- 848 Y Z/LConn3
  844 Y PQ/LConn3 -- 842-844 301/RConn3 -- 844/LConn3
  Ground12/LConn1 -- 858 Y PQ/RConn1
  864 Y PQ/RConn1 -- Ground11/LConn1
  820 Y PQ/RConn1 -- Ground5/LConn1
  844 Y PQ/LConn2 -- 842-844 301/RConn2 -- 844/LConn2
  Ground3/LConn1 -- 810 Y I/RConn1
  862 Y PQ/RConn1 -- Ground13/LConn1
  848 D PQ/LConn2 -- "848 "/RConn2 -- 848 Y Z/LConn2
  836-862 301/RConn1 -- 862/LConn1
  824 Y I/RConn1 -- Ground7/LConn1
  836-862 301/RConn2 -- 862/LConn2
  826 Y I/RConn1 -- Ground8/LConn1
  840/RConn3 -- 840 Y I/LConn3
  808 Y I/RConn1 -- Ground1/LConn1
  848 D PQ/LConn1 -- "848 "/RConn1 -- 848 Y Z/LConn1
  818 Y Z/RConn1 -- Ground2/LConn1
  844 Y PQ/LConn1 -- 842-844 301/RConn1 -- 844/LConn1
  822 Y PQ/RConn1 -- Ground6/LConn1
  860 Y PQ/LConn1 -- 860/RConn1 -- 860-836 301/LConn1 -- 860 D PQ/LConn1
  836 D PQ/LConn2 -- 860-836 301/RConn2 -- 836/LConn2
  860 D PQ/LConn3 -- 860-836 301/LConn3 -- 860/RConn3 -- 860 Y PQ/LConn3
  860 D PQ/LConn2 -- 860-836 301/LConn2 -- 860/RConn2 -- 860 Y PQ/LConn2
  840/RConn2 -- 840 Y I/LConn2
  836 D PQ/LConn3 -- 860-836 301/RConn3 -- 836/LConn3
  840/RConn1 -- 840 Y I/LConn1
  834 D Z/LConn3 -- 834/RConn3 -- 834-860 301/LConn3 -- 834-842 301/LConn3
  862 Y PQ/LConn1 -- 862-838 304/LConn1 -- 862/RConn2
  850-816 301/RConn1 -- "816 "/LConn1
  840 D I/LConn1 -- 836-840 301/RConn1 -- 840/LConn1
  854-852 301/RConn1 -- "852 "/LConn1
  834/LConn3 -- 858-834 301/RConn3 -- 834 D PQ/LConn3
  834 D PQ/LConn2 -- 858-834 301/RConn2 -- 834/LConn2
  854-852 301/RConn3 -- "852 "/LConn3
  834 D PQ/LConn1 -- 858-834 301/RConn1 -- 834/LConn1
  840 D I/LConn2 -- 836-840 301/RConn2 -- 840/LConn2
  858 D Z/LConn3 -- 858-834 301/LConn3 -- 858 D PQ/LConn3 -- 858/RConn3
  840 D I/LConn3 -- 836-840 301/RConn3 -- 840/LConn3
  854-852 301/LConn3 -- 854/RConn3
  854-852 301/LConn1 -- 854/RConn1
  854-852 301/RConn2 -- "852 "/LConn2
  850-816 301/RConn2 -- "816 "/LConn2
  850-816 301/RConn3 -- "816 "/LConn3
  854-856 303/LConn1 -- 854 Y PQ/LConn1 -- 854-852 301/LConn2 -- 854/RConn2
  836 D I/LConn2 -- 836-840 301/LConn2 -- 836-862 301/LConn2 -- 836/RConn2
  836 D I/LConn1 -- 836-840 301/LConn1 -- 836-862 301/LConn1 -- 836/RConn1
  848 Y PQ/LConn3 -- 846-848 301/RConn3 -- "848 "/LConn3
  846 Y PQ1/LConn3 -- 846-848 301/LConn3 -- 846/RConn3
  848 Y PQ/LConn2 -- 846-848 301/RConn2 -- "848 "/LConn2
  836 D I/LConn3 -- 836-840 301/LConn3 -- 836-862 301/LConn3 -- 836/RConn3
  848 Y PQ/LConn1 -- 846-848 301/RConn1 -- "848 "/LConn1
  846 Y PQ1/LConn2 -- 846-848 301/LConn2 -- 846/RConn2
  834/RConn2 -- 834 D Z/LConn2 -- 834-860 301/LConn2 -- 834-842 301/LConn2
  860 D Z/LConn3 -- 834-860 301/RConn3 -- 860/LConn3
  830-854 301/RConn1 -- 854/LConn1
  834-860 301/LConn1 -- 834-842 301/LConn1 -- 834/RConn1 -- 834 D Z/LConn1
  842 Y PQ/LConn3 -- 842-844 301/LConn3 -- 842/RConn3
  830-854 301/RConn2 -- 854/LConn2
  846 Y PQ1/LConn1 -- 846-848 301/LConn1 -- 846/RConn1
  832-858 301/RConn1 -- 858/LConn1
  844 Y PQ1/LConn3 -- 844-846 301/LConn3 -- 844/RConn3 -- 844 Y Z/LConn3 -- 844 Yg Z/LConn3
  842 Y PQ/LConn2 -- 842-844 301/LConn2 -- 842/RConn2
  844 Y PQ1/LConn1 -- 844-846 301/LConn1 -- 844/RConn1 -- 844 Yg Z/LConn1 -- 844 Y Z/LConn1
  832-858 301/RConn2 -- 858/LConn2
  830-854 301/RConn3 -- 854/LConn3
  842 Y PQ/LConn1 -- 842-844 301/LConn1 -- 842/RConn1
  860 D Z/LConn1 -- 834-860 301/RConn1 -- 860/LConn1
  830/RConn1 -- 830-854 301/LConn1 -- 830 D Z/LConn1
  830/RConn2 -- 830-854 301/LConn2 -- 830 D Z/LConn2
  846 Y PQ/LConn3 -- 844-846 301/RConn3 -- 846/LConn3
  846 Y PQ/LConn2 -- 844-846 301/RConn2 -- 846/LConn2
  832-858 301/RConn3 -- 858/LConn3
  844 Y PQ1/LConn2 -- 844-846 301/LConn2 -- 844/RConn2 -- 844 Yg Z/LConn2 -- 844 Y Z/LConn2
  830/RConn3 -- 830-854 301/LConn3 -- 830 D Z/LConn3
  860 D Z/LConn2 -- 834-860 301/RConn2 -- 860/LConn2
  846 Y PQ/LConn1 -- 844-846 301/RConn1 -- 846/LConn1
  818 Y Z/LConn1 -- 818-820 302/LConn1 -- 818/LConn1
  808-812 300/LConn3 -- 808/RConn3
  816 D I/LConn3 -- 816-824 301/LConn3 -- "816 "/RConn3
  806-808 300/RConn3 -- 808/LConn3
  816 D I/LConn1 -- "816 "/RConn1 -- 816-824 301/LConn1 -- 816-818 302/LConn1
  824 D I/LConn3 -- 816-824 301/RConn3 -- 824-828 301/LConn3 -- 824 Y PQ/LConn3 -- "824 "/LConn3
  808-812 300/LConn1 -- 808/RConn1
  806-808 300/RConn2 -- 808/LConn2
  824 Y I/LConn1 -- 824-826 303/LConn1 -- "824 "/RConn2
  828 Y PQ1/LConn2 -- 828-830 301/LConn2 -- 828/RConn2
  830 Y PQ/LConn2 -- 828-830 301/RConn2 -- 830/LConn2
  808 Y I/LConn1 -- 808-810 303/LConn1 -- 808-812 300/LConn2 -- 808/RConn2
  820/LConn1 -- 820-822 302/LConn1 -- 820 Y PQ/LConn1
  828 Y PQ1/LConn3 -- 828-830 301/LConn3 -- 828/RConn3
  "816 "/RConn2 -- 816-824 301/LConn2 -- 816 D I/LConn2
  828 Y PQ1/LConn1 -- 828-830 301/LConn1 -- 828/RConn1
  828 Y PQ/LConn2 -- 824-828 301/RConn2 -- 828/LConn2
  830 Y PQ/LConn3 -- 828-830 301/RConn3 -- 830/LConn3
  828 Y PQ/LConn1 -- 824-828 301/RConn1 -- 828/LConn1
  816-824 301/RConn2 -- 824 D I/LConn2 -- 824-828 301/LConn2 -- 824 Y PQ/LConn2 -- "824 "/LConn2
  830 Y PQ/LConn1 -- 828-830 301/RConn1 -- 830/LConn1
  828 Y PQ/LConn3 -- 824-828 301/RConn3 -- 828/LConn3
  824 D I/LConn1 -- 816-824 301/RConn1 -- 824-828 301/LConn1 -- 824 Y PQ/LConn1 -- "824 "/LConn1
  802-806 300/RConn1 -- 806/LConn1
  802 Y PQ/LConn3 -- 802-806 300/LConn3 -- 802/RConn3
  800-802 300/RConn2 -- 802/LConn2
  806 Y PQ/LConn2 -- 806-808 300/LConn2 -- 806/RConn2
  806 Y PQ/LConn1 -- 806-808 300/LConn1 -- 806/RConn1
  802-806 300/RConn3 -- 806/LConn3
  802 Y PQ/LConn1 -- 802-806 300/LConn1 -- 802/RConn1
  806-808 300/RConn1 -- 808/LConn1
  800-802 300/RConn3 -- 802/LConn3
  802 Y PQ/LConn2 -- 802-806 300/LConn2 -- 802/RConn2
  806 Y PQ/LConn3 -- 806-808 300/LConn3 -- 806/RConn3
  802-806 300/RConn2 -- 806/LConn2
  800-802 300/RConn1 -- 802/LConn1
  Regulator 1/LConn1 -- 814/RConn1
  Regulator 1/LConn2 -- 814/RConn2
  Regulator 1/LConn3 -- 814/RConn3
  Regulator 1/RConn1 -- RG10/LConn1
  Regulator 1/RConn2 -- RG10/LConn2
  Regulator 1/RConn3 -- RG10/LConn3
  Regulator 2/LConn1 -- "852 "/RConn1
  Regulator 2/LConn2 -- "852 "/RConn2
  Regulator 2/LConn3 -- "852 "/RConn3
  Regulator 2/RConn1 -- RG11/LConn1
  RG11/LConn2 -- Regulator 2/RConn2
  RG11/LConn3 -- Regulator 2/RConn3
